simulink model "SUB_IoControl"  (R2018b)
settings: Solver=VariableStepDiscrete  StartTime=0.0  StopTime=10  RelTol=1e-3
PreLoadFcn:
  | if(exist('MBDS_ModelCallback', 'file'))
  |    MBDS_ModelCallback('PreLoad');
  | end
PostLoadFcn:
  | if(exist('MBDS_ModelCallback', 'file'))
  |    MBDS_ModelCallback('PostLoad');
  | end
InitFcn:
  | if(exist('MBDS_ModelCallback', 'file'))
  |    MBDS_ModelCallback('Init');
  | end
StartFcn:
  | if(exist('MBDS_ModelCallback', 'file'))
  |    MBDS_ModelCallback('Start');
  | end
StopFcn:
  | if(exist('MBDS_ModelCallback', 'file'))
  |    MBDS_ModelCallback('Stop');
  | end
undefined symbols (not defined in the file): sigbuilder_block
libraries: KIBES_Signal x742, MBDS_Modules x38, simulink x1
(part 7 of 8)

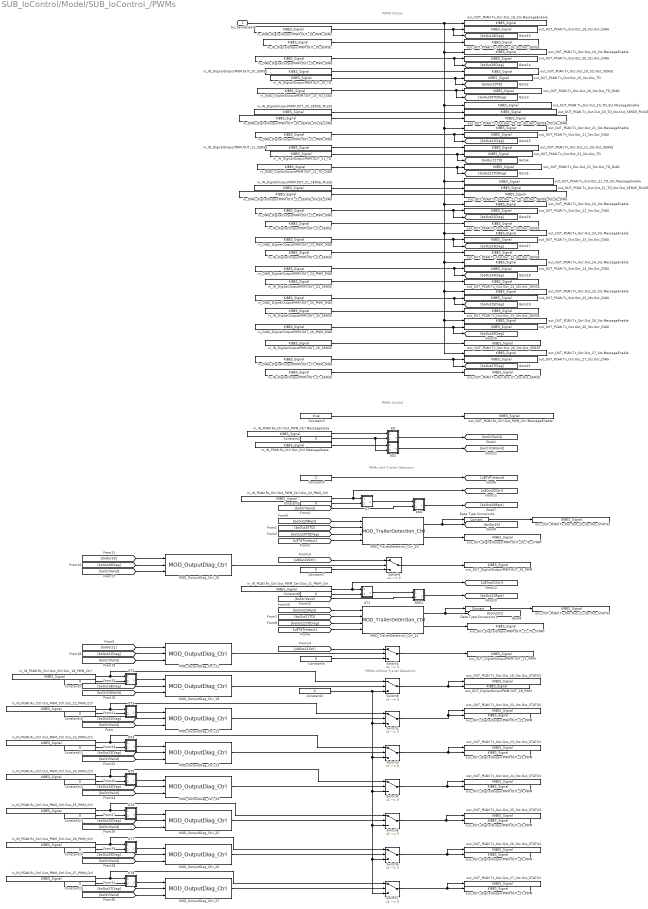
== system SUB_IoControl/Model/SUB_IoControl_/PWMs ==
  note: PWMs Control
  note: PWMs Status
  note: PWMs with Trailer Detection
  note: PWMs without Trailer Detection
  bo_SendEnable : Inport
  AND : Subsystem  InitFcn=|  mask(AND){MBDS_LibraryBlock=on, BitwiseMode=off, Inputs=2, UseBitMask=off, BitMask='A7', OutDataTypeStr=Inherit: Inherit via back propagation, MBDS_BlockVersion=08.20.02}
      | if(exist('MBDS_BlockCallback', 'file'))
      |    MBDS_BlockCallback('Update', gcb);
      | end
      mask prompts: MBDS_LibraryBlock "MBDS library block"; BitwiseMode "Use 'bitwise' mode"; Inputs "Number of input ports:"; UseBitMask "Use bit mask"; BitMask "Bit mask:"; OutDataTypeStr "Output data type:"; MBDS_BlockVersion "Version:"
      mask help: Logical or bitwise AND operator. For multiple inputs, operators are applied across the inputs. For a single input, operators are applied across the input vector. In bitwise mode a bit mask can be applied onto single input signals.
      mask init: same as SUB_IoControl/Outputs/AnalyseOutputs/And
      mask Help: eval(['open([workdir(''library_dir:''),''\Blockset\help\'',get_param(gcb,''MaskType''),''.html''])'])
      mask Callback BitwiseMode:
      | if(exist('MBDS_BlockCallback', 'file'))
      |    MBDS_BlockCallback('BitwiseMode', gcb);
      | end
      mask Callback Inputs:
      | if(exist('MBDS_BlockCallback', 'file'))
      |    MBDS_BlockCallback('Inputs', gcb);
      | end
      mask Callback UseBitMask:
      | if(exist('MBDS_BlockCallback', 'file'))
      |    MBDS_BlockCallback('UseBitMask', gcb);
      | end
      mask Callback BitMask:
      | if(exist('MBDS_BlockCallback', 'file'))
      |    MBDS_BlockCallback('BitMask', gcb);
      | end
      mask TypeOptions OutDataTypeStr: Inherit: Inherit via back propagation | int8 | uint8 | int16 | uint16 | int32 | uint32 | boolean
      mask Callback OutDataTypeStr:
      | % Adopt Value
      | if(exist('MBDS_BlockCallback', 'file'))
      |    MBDS_BlockCallback('OutDataTypeStr', gcb);
      | end
      mask DialogControl ParameterTabVar0 Prompt: Main
      mask DialogControl ParameterTabVar01 Prompt: Signal Attributes
      mask DialogControl ParameterTabVar012 Prompt: Version
      mask Display:
      | % Show icon or block text
      | if(UseBitMask)
      |    if(isnumeric(BitMask))
      |       BitMaskString = ['0x',dec2hex(floor(BitMask))];
      |    elseif(ischar(BitMask))
      |       BitMaskString = ['0x',upper(BitMask)];
      |    else
      |       BitMaskString = '???';
      |    end
      |    disp(sprintf(['AND\n', BitMaskString]))
      | else
      |    disp('AND')
      | end
  AND1 : Subsystem  InitFcn=|  mask(AND){MBDS_LibraryBlock=on, BitwiseMode=off, Inputs=2, UseBitMask=off, BitMask='A7', OutDataTypeStr=Inherit: Inherit via back propagation, MBDS_BlockVersion=08.20.02}
      | if(exist('MBDS_BlockCallback', 'file'))
      |    MBDS_BlockCallback('Update', gcb);
      | end
      mask prompts: MBDS_LibraryBlock "MBDS library block"; BitwiseMode "Use 'bitwise' mode"; Inputs "Number of input ports:"; UseBitMask "Use bit mask"; BitMask "Bit mask:"; OutDataTypeStr "Output data type:"; MBDS_BlockVersion "Version:"
      mask help: Logical or bitwise AND operator. For multiple inputs, operators are applied across the inputs. For a single input, operators are applied across the input vector. In bitwise mode a bit mask can be applied onto single input signals.
      mask init: same as SUB_IoControl/Outputs/AnalyseOutputs/And
      mask Help: eval(['open([workdir(''library_dir:''),''\Blockset\help\'',get_param(gcb,''MaskType''),''.html''])'])
      mask Callback BitwiseMode:
      | if(exist('MBDS_BlockCallback', 'file'))
      |    MBDS_BlockCallback('BitwiseMode', gcb);
      | end
      mask Callback Inputs:
      | if(exist('MBDS_BlockCallback', 'file'))
      |    MBDS_BlockCallback('Inputs', gcb);
      | end
      mask Callback UseBitMask:
      | if(exist('MBDS_BlockCallback', 'file'))
      |    MBDS_BlockCallback('UseBitMask', gcb);
      | end
      mask Callback BitMask:
      | if(exist('MBDS_BlockCallback', 'file'))
      |    MBDS_BlockCallback('BitMask', gcb);
      | end
      mask TypeOptions OutDataTypeStr: Inherit: Inherit via back propagation | int8 | uint8 | int16 | uint16 | int32 | uint32 | boolean
      mask Callback OutDataTypeStr:
      | % Adopt Value
      | if(exist('MBDS_BlockCallback', 'file'))
      |    MBDS_BlockCallback('OutDataTypeStr', gcb);
      | end
      mask DialogControl ParameterTabVar0 Prompt: Main
      mask DialogControl ParameterTabVar01 Prompt: Signal Attributes
      mask DialogControl ParameterTabVar012 Prompt: Version
      mask Display:
      | % Show icon or block text
      | if(UseBitMask)
      |    if(isnumeric(BitMask))
      |       BitMaskString = ['0x',dec2hex(floor(BitMask))];
      |    elseif(ischar(BitMask))
      |       BitMaskString = ['0x',upper(BitMask)];
      |    else
      |       BitMaskString = '???';
      |    end
      |    disp(sprintf(['AND\n', BitMaskString]))
      | else
      |    disp('AND')
      | end
  Constant1 : Constant  InitFcn=|  Value=0  OutDataTypeStr=uint16
      | if(exist('MBDS_BlockCallback', 'file'))
      |    MBDS_BlockCallback('Update', gcb);  
      | end
  Constant10 : Constant  InitFcn=|  Value=0  OutDataTypeStr=uint8
      | if(exist('MBDS_BlockCallback', 'file'))
      |    MBDS_BlockCallback('Update', gcb);  
      | end
  Constant11 : Constant  InitFcn=|  Value=0  OutDataTypeStr=uint8
      | if(exist('MBDS_BlockCallback', 'file'))
      |    MBDS_BlockCallback('Update', gcb);  
      | end
  Constant12 : Constant  InitFcn=|  Value=0  OutDataTypeStr=uint8
      | if(exist('MBDS_BlockCallback', 'file'))
      |    MBDS_BlockCallback('Update', gcb);  
      | end
  Constant13 : Constant  InitFcn=|  Value=0  OutDataTypeStr=uint8
      | if(exist('MBDS_BlockCallback', 'file'))
      |    MBDS_BlockCallback('Update', gcb);  
      | end
  Constant14 : Constant  InitFcn=|  Value=0  OutDataTypeStr=uint8
      | if(exist('MBDS_BlockCallback', 'file'))
      |    MBDS_BlockCallback('Update', gcb);  
      | end
  Constant15 : Constant  InitFcn=|  Value=0  OutDataTypeStr=uint8
      | if(exist('MBDS_BlockCallback', 'file'))
      |    MBDS_BlockCallback('Update', gcb);  
      | end
  Constant2 : Constant  InitFcn=|  Value=0  OutDataTypeStr=uint16
      | if(exist('MBDS_BlockCallback', 'file'))
      |    MBDS_BlockCallback('Update', gcb);  
      | end
  Constant3 : Constant  InitFcn=|  Value=true  OutDataTypeStr=boolean
      | if(exist('MBDS_BlockCallback', 'file'))
      |    MBDS_BlockCallback('Update', gcb);  
      | end
  Constant4 : Constant  InitFcn=|  Value=2  OutDataTypeStr=uint8
      | if(exist('MBDS_BlockCallback', 'file'))
      |    MBDS_BlockCallback('Update', gcb);  
      | end
  Constant5 : Constant  InitFcn=|  Value=0  OutDataTypeStr=uint8
      | if(exist('MBDS_BlockCallback', 'file'))
      |    MBDS_BlockCallback('Update', gcb);  
      | end
  Constant6 : Constant  InitFcn=|  Value=0  OutDataTypeStr=uint16
      | if(exist('MBDS_BlockCallback', 'file'))
      |    MBDS_BlockCallback('Update', gcb);  
      | end
  Constant7 : Constant  InitFcn=|  Value=0  OutDataTypeStr=uint8
      | if(exist('MBDS_BlockCallback', 'file'))
      |    MBDS_BlockCallback('Update', gcb);  
      | end
  Constant8 : Constant  InitFcn=|  Value=0  OutDataTypeStr=uint8
      | if(exist('MBDS_BlockCallback', 'file'))
      |    MBDS_BlockCallback('Update', gcb);  
      | end
  Constant9 : Constant  InitFcn=|  Value=0  OutDataTypeStr=uint8
      | if(exist('MBDS_BlockCallback', 'file'))
      |    MBDS_BlockCallback('Update', gcb);  
      | end
  Data Type Conversion : DataTypeConversion  InitFcn=|  SaturateOnIntegerOverflow=on
      | try
      |    MBDS_BlockCallback('Update', gcb);
      | end
      settings: AttributesFormatString=Saturate: %<SaturateOnIntegerOverflow>
  Data Type Conversion1 : DataTypeConversion  InitFcn=|  SaturateOnIntegerOverflow=on
      | try
      |    MBDS_BlockCallback('Update', gcb);
      | end
      settings: AttributesFormatString=Saturate: %<SaturateOnIntegerOverflow>
  EQ : Subsystem  InitFcn=|  mask(EQ){MBDS_LibraryBlock=on, InputSameDT=on, MBDS_BlockVersion=08.20.02}
      | if(exist('MBDS_BlockCallback', 'file'))
      |    MBDS_BlockCallback('Update', gcb);
      | end
      mask prompts: MBDS_LibraryBlock "MBDS library block"; InputSameDT "Require all inputs to have the same data type"; MBDS_BlockVersion "Block version:"
      mask help: The block compares if both input signals are equal.
      mask init: same as SUB_IoControl/Outputs/AnalyseOutputs/And
      mask Help: eval(['open([workdir(''library_dir:''),''\Blockset\help\'',get_param(gcb,''MaskType''),''.html''])'])
      mask Callback InputSameDT:
      | % Adopt value
      | if(exist('MBDS_BlockCallback', 'file'))
      |    MBDS_BlockCallback('InputSameDT', gcb);
      | end
      mask DialogControl ParameterTabVar0 Prompt: Signal Attributes
      mask DialogControl ParameterTabVar01 Prompt: Version
      mask Display:
      | % Show icon or block text
      | if(exist('MBDS_BlockCallback', 'file'))
      |    image(imread('EQ.tif','tif'),[0.35,0.35,0.355,0.25])
      |    disp('')
      | else
      |    disp(sprintf('=='));
      | end
  EQ1 : Subsystem  InitFcn=|  mask(EQ){MBDS_LibraryBlock=on, InputSameDT=on, MBDS_BlockVersion=08.20.02}
      | if(exist('MBDS_BlockCallback', 'file'))
      |    MBDS_BlockCallback('Update', gcb);
      | end
      mask prompts: MBDS_LibraryBlock "MBDS library block"; InputSameDT "Require all inputs to have the same data type"; MBDS_BlockVersion "Block version:"
      mask help: The block compares if both input signals are equal.
      mask init: same as SUB_IoControl/Outputs/AnalyseOutputs/And
      mask Help: eval(['open([workdir(''library_dir:''),''\Blockset\help\'',get_param(gcb,''MaskType''),''.html''])'])
      mask Callback InputSameDT:
      | % Adopt value
      | if(exist('MBDS_BlockCallback', 'file'))
      |    MBDS_BlockCallback('InputSameDT', gcb);
      | end
      mask DialogControl ParameterTabVar0 Prompt: Signal Attributes
      mask DialogControl ParameterTabVar01 Prompt: Version
      mask Display:
      | % Show icon or block text
      | if(exist('MBDS_BlockCallback', 'file'))
      |    image(imread('EQ.tif','tif'),[0.35,0.35,0.355,0.25])
      |    disp('')
      | else
      |    disp(sprintf('=='));
      | end
  GT : Subsystem  InitFcn=|  mask(GT){MBDS_LibraryBlock=on, InputSameDT=on, MBDS_BlockVersion=08.20.02}
      | if(exist('MBDS_BlockCallback', 'file'))
      |    MBDS_BlockCallback('Update', gcb);
      | end
      mask prompts: MBDS_LibraryBlock "MBDS library block"; InputSameDT "Require all inputs to have the same data type"; MBDS_BlockVersion "Block version:"
      mask help: The block compares if the first input signal is greater than the second input signal.
      mask init: same as SUB_IoControl/Outputs/AnalyseOutputs/And
      mask Help: eval(['open([workdir(''library_dir:''),''\Blockset\help\'',get_param(gcb,''MaskType''),''.html''])'])
      mask Callback InputSameDT:
      | % Adopt value
      | if(exist('MBDS_BlockCallback', 'file'))
      |    MBDS_BlockCallback('InputSameDT', gcb);
      | end
      mask DialogControl ParameterTabVar0 Prompt: Signal Attributes
      mask DialogControl ParameterTabVar01 Prompt: Version
      mask Display:
      | % Show icon or block text
      | if(exist('MBDS_BlockCallback', 'file'))
      |    image(imread('GT.tif','tif'),[0.33,0.33,0.37,0.37])
      |    disp('')
      | else
      |    disp(sprintf('>'));
      | end
  GT1 : Subsystem  InitFcn=|  mask(GT){MBDS_LibraryBlock=on, InputSameDT=on, MBDS_BlockVersion=08.20.02}
      | if(exist('MBDS_BlockCallback', 'file'))
      |    MBDS_BlockCallback('Update', gcb);
      | end
      mask prompts: MBDS_LibraryBlock "MBDS library block"; InputSameDT "Require all inputs to have the same data type"; MBDS_BlockVersion "Block version:"
      mask help: The block compares if the first input signal is greater than the second input signal.
      mask init: same as SUB_IoControl/Outputs/AnalyseOutputs/And
      mask Help: eval(['open([workdir(''library_dir:''),''\Blockset\help\'',get_param(gcb,''MaskType''),''.html''])'])
      mask Callback InputSameDT:
      | % Adopt value
      | if(exist('MBDS_BlockCallback', 'file'))
      |    MBDS_BlockCallback('InputSameDT', gcb);
      | end
      mask DialogControl ParameterTabVar0 Prompt: Signal Attributes
      mask DialogControl ParameterTabVar01 Prompt: Version
      mask Display:
      | % Show icon or block text
      | if(exist('MBDS_BlockCallback', 'file'))
      |    image(imread('GT.tif','tif'),[0.33,0.33,0.37,0.37])
      |    disp('')
      | else
      |    disp(sprintf('>'));
      | end
  GT2 : Subsystem  InitFcn=|  mask(GT){MBDS_LibraryBlock=on, InputSameDT=on, MBDS_BlockVersion=08.20.02}
      | if(exist('MBDS_BlockCallback', 'file'))
      |    MBDS_BlockCallback('Update', gcb);
      | end
      mask prompts: MBDS_LibraryBlock "MBDS library block"; InputSameDT "Require all inputs to have the same data type"; MBDS_BlockVersion "Block version:"
      mask help: The block compares if the first input signal is greater than the second input signal.
      mask init: same as SUB_IoControl/Outputs/AnalyseOutputs/And
      mask Help: eval(['open([workdir(''library_dir:''),''\Blockset\help\'',get_param(gcb,''MaskType''),''.html''])'])
      mask Callback InputSameDT:
      | % Adopt value
      | if(exist('MBDS_BlockCallback', 'file'))
      |    MBDS_BlockCallback('InputSameDT', gcb);
      | end
      mask DialogControl ParameterTabVar0 Prompt: Signal Attributes
      mask DialogControl ParameterTabVar01 Prompt: Version
      mask Display:
      | % Show icon or block text
      | if(exist('MBDS_BlockCallback', 'file'))
      |    image(imread('GT.tif','tif'),[0.33,0.33,0.37,0.37])
      |    disp('')
      | else
      |    disp(sprintf('>'));
      | end
  GT3 : Subsystem  InitFcn=|  mask(GT){MBDS_LibraryBlock=on, InputSameDT=on, MBDS_BlockVersion=08.20.02}
      | if(exist('MBDS_BlockCallback', 'file'))
      |    MBDS_BlockCallback('Update', gcb);
      | end
      mask prompts: MBDS_LibraryBlock "MBDS library block"; InputSameDT "Require all inputs to have the same data type"; MBDS_BlockVersion "Block version:"
      mask help: The block compares if the first input signal is greater than the second input signal.
      mask init: same as SUB_IoControl/Outputs/AnalyseOutputs/And
      mask Help: eval(['open([workdir(''library_dir:''),''\Blockset\help\'',get_param(gcb,''MaskType''),''.html''])'])
      mask Callback InputSameDT:
      | % Adopt value
      | if(exist('MBDS_BlockCallback', 'file'))
      |    MBDS_BlockCallback('InputSameDT', gcb);
      | end
      mask DialogControl ParameterTabVar0 Prompt: Signal Attributes
      mask DialogControl ParameterTabVar01 Prompt: Version
      mask Display:
      | % Show icon or block text
      | if(exist('MBDS_BlockCallback', 'file'))
      |    image(imread('GT.tif','tif'),[0.33,0.33,0.37,0.37])
      |    disp('')
      | else
      |    disp(sprintf('>'));
      | end
  GT4 : Subsystem  InitFcn=|  mask(GT){MBDS_LibraryBlock=on, InputSameDT=on, MBDS_BlockVersion=08.20.02}
      | if(exist('MBDS_BlockCallback', 'file'))
      |    MBDS_BlockCallback('Update', gcb);
      | end
      mask prompts: MBDS_LibraryBlock "MBDS library block"; InputSameDT "Require all inputs to have the same data type"; MBDS_BlockVersion "Block version:"
      mask help: The block compares if the first input signal is greater than the second input signal.
      mask init: same as SUB_IoControl/Outputs/AnalyseOutputs/And
      mask Help: eval(['open([workdir(''library_dir:''),''\Blockset\help\'',get_param(gcb,''MaskType''),''.html''])'])
      mask Callback InputSameDT:
      | % Adopt value
      | if(exist('MBDS_BlockCallback', 'file'))
      |    MBDS_BlockCallback('InputSameDT', gcb);
      | end
      mask DialogControl ParameterTabVar0 Prompt: Signal Attributes
      mask DialogControl ParameterTabVar01 Prompt: Version
      mask Display:
      | % Show icon or block text
      | if(exist('MBDS_BlockCallback', 'file'))
      |    image(imread('GT.tif','tif'),[0.33,0.33,0.37,0.37])
      |    disp('')
      | else
      |    disp(sprintf('>'));
      | end
  GT5 : Subsystem  InitFcn=|  mask(GT){MBDS_LibraryBlock=on, InputSameDT=on, MBDS_BlockVersion=08.20.02}
      | if(exist('MBDS_BlockCallback', 'file'))
      |    MBDS_BlockCallback('Update', gcb);
      | end
      mask prompts: MBDS_LibraryBlock "MBDS library block"; InputSameDT "Require all inputs to have the same data type"; MBDS_BlockVersion "Block version:"
      mask help: The block compares if the first input signal is greater than the second input signal.
      mask init: same as SUB_IoControl/Outputs/AnalyseOutputs/And
      mask Help: eval(['open([workdir(''library_dir:''),''\Blockset\help\'',get_param(gcb,''MaskType''),''.html''])'])
      mask Callback InputSameDT:
      | % Adopt value
      | if(exist('MBDS_BlockCallback', 'file'))
      |    MBDS_BlockCallback('InputSameDT', gcb);
      | end
      mask DialogControl ParameterTabVar0 Prompt: Signal Attributes
      mask DialogControl ParameterTabVar01 Prompt: Version
      mask Display:
      | % Show icon or block text
      | if(exist('MBDS_BlockCallback', 'file'))
      |    image(imread('GT.tif','tif'),[0.33,0.33,0.37,0.37])
      |    disp('')
      | else
      |    disp(sprintf('>'));
      | end
  GT6 : Subsystem  InitFcn=|  mask(GT){MBDS_LibraryBlock=on, InputSameDT=on, MBDS_BlockVersion=08.20.02}
      | if(exist('MBDS_BlockCallback', 'file'))
      |    MBDS_BlockCallback('Update', gcb);
      | end
      mask prompts: MBDS_LibraryBlock "MBDS library block"; InputSameDT "Require all inputs to have the same data type"; MBDS_BlockVersion "Block version:"
      mask help: The block compares if the first input signal is greater than the second input signal.
      mask init: same as SUB_IoControl/Outputs/AnalyseOutputs/And
      mask Help: eval(['open([workdir(''library_dir:''),''\Blockset\help\'',get_param(gcb,''MaskType''),''.html''])'])
      mask Callback InputSameDT:
      | % Adopt value
      | if(exist('MBDS_BlockCallback', 'file'))
      |    MBDS_BlockCallback('InputSameDT', gcb);
      | end
      mask DialogControl ParameterTabVar0 Prompt: Signal Attributes
      mask DialogControl ParameterTabVar01 Prompt: Version
      mask Display:
      | % Show icon or block text
      | if(exist('MBDS_BlockCallback', 'file'))
      |    image(imread('GT.tif','tif'),[0.33,0.33,0.37,0.37])
      |    disp('')
      | else
      |    disp(sprintf('>'));
      | end
  GT7 : Subsystem  InitFcn=|  mask(GT){MBDS_LibraryBlock=on, InputSameDT=on, MBDS_BlockVersion=08.20.02}
      | if(exist('MBDS_BlockCallback', 'file'))
      |    MBDS_BlockCallback('Update', gcb);
      | end
      mask prompts: MBDS_LibraryBlock "MBDS library block"; InputSameDT "Require all inputs to have the same data type"; MBDS_BlockVersion "Block version:"
      mask help: The block compares if the first input signal is greater than the second input signal.
      mask init: same as SUB_IoControl/Outputs/AnalyseOutputs/And
      mask Help: eval(['open([workdir(''library_dir:''),''\Blockset\help\'',get_param(gcb,''MaskType''),''.html''])'])
      mask Callback InputSameDT:
      | % Adopt value
      | if(exist('MBDS_BlockCallback', 'file'))
      |    MBDS_BlockCallback('InputSameDT', gcb);
      | end
      mask DialogControl ParameterTabVar0 Prompt: Signal Attributes
      mask DialogControl ParameterTabVar01 Prompt: Version
      mask Display:
      | % Show icon or block text
      | if(exist('MBDS_BlockCallback', 'file'))
      |    image(imread('GT.tif','tif'),[0.33,0.33,0.37,0.37])
      |    disp('')
      | else
      |    disp(sprintf('>'));
      | end
  GT8 : Subsystem  InitFcn=|  mask(GT){MBDS_LibraryBlock=on, InputSameDT=on, MBDS_BlockVersion=08.20.02}
      | if(exist('MBDS_BlockCallback', 'file'))
      |    MBDS_BlockCallback('Update', gcb);
      | end
      mask prompts: MBDS_LibraryBlock "MBDS library block"; InputSameDT "Require all inputs to have the same data type"; MBDS_BlockVersion "Block version:"
      mask help: The block compares if the first input signal is greater than the second input signal.
      mask init: same as SUB_IoControl/Outputs/AnalyseOutputs/And
      mask Help: eval(['open([workdir(''library_dir:''),''\Blockset\help\'',get_param(gcb,''MaskType''),''.html''])'])
      mask Callback InputSameDT:
      | % Adopt value
      | if(exist('MBDS_BlockCallback', 'file'))
      |    MBDS_BlockCallback('InputSameDT', gcb);
      | end
      mask DialogControl ParameterTabVar0 Prompt: Signal Attributes
      mask DialogControl ParameterTabVar01 Prompt: Version
      mask Display:
      | % Show icon or block text
      | if(exist('MBDS_BlockCallback', 'file'))
      |    image(imread('GT.tif','tif'),[0.33,0.33,0.37,0.37])
      |    disp('')
      | else
      |    disp(sprintf('>'));
      | end
  MOD_OutputDiag_Ctrl_{18,20..27} (9 alike) : MBDS_Modules/MOD_OutputDiag_Ctrl  Description=Controls output based on diagnostic signal  MBDS_ElementType=Module  MBDS_WorkStatus=In Work  MBDS_LastModified=2021-03-24-14:11:54
      settings: SourceProductName=MBDS Project Library
  MOD_TrailerDetection_Ctrl_20 : MBDS_Modules/MOD_TrailerDetection_Ctrl  Description=Control outputs with Trailer detection hardware.  MBDS_ElementType=Module  MBDS_WorkStatus=In Work  MBDS_LastModified=2020-12-28-09:09:43
      settings: SourceProductName=MBDS Project Library
  MOD_TrailerDetection_Ctrl_21 : MBDS_Modules/MOD_TrailerDetection_Ctrl  Description=Control outputs with Trailer detection hardware.  MBDS_ElementType=Module  MBDS_WorkStatus=In Work  MBDS_LastModified=2020-12-28-09:09:43
      settings: SourceProductName=MBDS Project Library
  Switch1 : Switch  InitFcn=|  Criteria=u2 ~= 0  OutDataTypeStr=Inherit: Inherit via back propagation  mask(Switch){MBDS_LibraryBlock=on, OutDataTypeStr_=Inherit: Inherit via back propagation, SaturateOnIntegerOverflow_=off, InputSameDT_=off, MBDS_BlockVersion=08.20.02}
      | if(exist('MBDS_BlockCallback', 'file'))
      |    MBDS_BlockCallback('Update', gcb);  
      | end
      mask prompts: MBDS_LibraryBlock "MBDS library block"; OutDataTypeStr_ "Output data type:"; SaturateOnIntegerOverflow_ "Saturate on integer overflow"; InputSameDT_ "Require all inputs to have the same data type"; MBDS_BlockVersion "Block version:"
      mask help: Pass through input 1 when input 2 is not equal to zero; otherwise pass through input 3. The inputs are numbered top to bottom (or left to right). The first and third input ports are data ports, and the second input port is the control port.
      mask init: same as SUB_IoControl/Outputs/AnalyseOutputs/And
      mask Help: eval(['open([workdir(''library_dir:''),''\Blockset\help\'',get_param(gcb,''MaskType''),''.html''])'])
      mask TypeOptions OutDataTypeStr_: Inherit: Inherit via back propagation | single | int8 | uint8 | int16 | uint16 | int32 | uint32
      mask DialogControl ParameterTabVar0 Prompt: Signal Attributes
      mask DialogControl ParameterTabVar01 Prompt: Version
  Switch2 : Switch  InitFcn=|  Criteria=u2 ~= 0  OutDataTypeStr=Inherit: Inherit via back propagation  mask(Switch){MBDS_LibraryBlock=on, OutDataTypeStr_=Inherit: Inherit via back propagation, SaturateOnIntegerOverflow_=off, InputSameDT_=off, MBDS_BlockVersion=08.20.02}
      | if(exist('MBDS_BlockCallback', 'file'))
      |    MBDS_BlockCallback('Update', gcb);  
      | end
      mask prompts: MBDS_LibraryBlock "MBDS library block"; OutDataTypeStr_ "Output data type:"; SaturateOnIntegerOverflow_ "Saturate on integer overflow"; InputSameDT_ "Require all inputs to have the same data type"; MBDS_BlockVersion "Block version:"
      mask help: Pass through input 1 when input 2 is not equal to zero; otherwise pass through input 3. The inputs are numbered top to bottom (or left to right). The first and third input ports are data ports, and the second input port is the control port.
      mask init: same as SUB_IoControl/Outputs/AnalyseOutputs/And
      mask Help: eval(['open([workdir(''library_dir:''),''\Blockset\help\'',get_param(gcb,''MaskType''),''.html''])'])
      mask TypeOptions OutDataTypeStr_: Inherit: Inherit via back propagation | single | int8 | uint8 | int16 | uint16 | int32 | uint32
      mask DialogControl ParameterTabVar0 Prompt: Signal Attributes
      mask DialogControl ParameterTabVar01 Prompt: Version
  Switch3 : Switch  InitFcn=|  Criteria=u2 ~= 0  OutDataTypeStr=Inherit: Inherit via back propagation  mask(Switch){MBDS_LibraryBlock=on, OutDataTypeStr_=Inherit: Inherit via back propagation, SaturateOnIntegerOverflow_=off, InputSameDT_=off, MBDS_BlockVersion=08.20.02}
      | if(exist('MBDS_BlockCallback', 'file'))
      |    MBDS_BlockCallback('Update', gcb);  
      | end
      mask prompts: MBDS_LibraryBlock "MBDS library block"; OutDataTypeStr_ "Output data type:"; SaturateOnIntegerOverflow_ "Saturate on integer overflow"; InputSameDT_ "Require all inputs to have the same data type"; MBDS_BlockVersion "Block version:"
      mask help: Pass through input 1 when input 2 is not equal to zero; otherwise pass through input 3. The inputs are numbered top to bottom (or left to right). The first and third input ports are data ports, and the second input port is the control port.
      mask init: same as SUB_IoControl/Outputs/AnalyseOutputs/And
      mask Help: eval(['open([workdir(''library_dir:''),''\Blockset\help\'',get_param(gcb,''MaskType''),''.html''])'])
      mask TypeOptions OutDataTypeStr_: Inherit: Inherit via back propagation | single | int8 | uint8 | int16 | uint16 | int32 | uint32
      mask DialogControl ParameterTabVar0 Prompt: Signal Attributes
      mask DialogControl ParameterTabVar01 Prompt: Version
  Switch4 : Switch  InitFcn=|  Criteria=u2 ~= 0  OutDataTypeStr=Inherit: Inherit via back propagation  mask(Switch){MBDS_LibraryBlock=on, OutDataTypeStr_=Inherit: Inherit via back propagation, SaturateOnIntegerOverflow_=off, InputSameDT_=off, MBDS_BlockVersion=08.20.02}
      | if(exist('MBDS_BlockCallback', 'file'))
      |    MBDS_BlockCallback('Update', gcb);  
      | end
      mask prompts: MBDS_LibraryBlock "MBDS library block"; OutDataTypeStr_ "Output data type:"; SaturateOnIntegerOverflow_ "Saturate on integer overflow"; InputSameDT_ "Require all inputs to have the same data type"; MBDS_BlockVersion "Block version:"
      mask help: Pass through input 1 when input 2 is not equal to zero; otherwise pass through input 3. The inputs are numbered top to bottom (or left to right). The first and third input ports are data ports, and the second input port is the control port.
      mask init: same as SUB_IoControl/Outputs/AnalyseOutputs/And
      mask Help: eval(['open([workdir(''library_dir:''),''\Blockset\help\'',get_param(gcb,''MaskType''),''.html''])'])
      mask TypeOptions OutDataTypeStr_: Inherit: Inherit via back propagation | single | int8 | uint8 | int16 | uint16 | int32 | uint32
      mask DialogControl ParameterTabVar0 Prompt: Signal Attributes
      mask DialogControl ParameterTabVar01 Prompt: Version
  Switch5 : Switch  InitFcn=|  Criteria=u2 ~= 0  OutDataTypeStr=Inherit: Inherit via back propagation  mask(Switch){MBDS_LibraryBlock=on, OutDataTypeStr_=Inherit: Inherit via back propagation, SaturateOnIntegerOverflow_=off, InputSameDT_=off, MBDS_BlockVersion=08.20.02}
      | if(exist('MBDS_BlockCallback', 'file'))
      |    MBDS_BlockCallback('Update', gcb);  
      | end
      mask prompts: MBDS_LibraryBlock "MBDS library block"; OutDataTypeStr_ "Output data type:"; SaturateOnIntegerOverflow_ "Saturate on integer overflow"; InputSameDT_ "Require all inputs to have the same data type"; MBDS_BlockVersion "Block version:"
      mask help: Pass through input 1 when input 2 is not equal to zero; otherwise pass through input 3. The inputs are numbered top to bottom (or left to right). The first and third input ports are data ports, and the second input port is the control port.
      mask init: same as SUB_IoControl/Outputs/AnalyseOutputs/And
      mask Help: eval(['open([workdir(''library_dir:''),''\Blockset\help\'',get_param(gcb,''MaskType''),''.html''])'])
      mask TypeOptions OutDataTypeStr_: Inherit: Inherit via back propagation | single | int8 | uint8 | int16 | uint16 | int32 | uint32
      mask DialogControl ParameterTabVar0 Prompt: Signal Attributes
      mask DialogControl ParameterTabVar01 Prompt: Version
  Switch6 : Switch  InitFcn=|  Criteria=u2 ~= 0  OutDataTypeStr=Inherit: Inherit via back propagation  mask(Switch){MBDS_LibraryBlock=on, OutDataTypeStr_=Inherit: Inherit via back propagation, SaturateOnIntegerOverflow_=off, InputSameDT_=off, MBDS_BlockVersion=08.20.02}
      | if(exist('MBDS_BlockCallback', 'file'))
      |    MBDS_BlockCallback('Update', gcb);  
      | end
      mask prompts: MBDS_LibraryBlock "MBDS library block"; OutDataTypeStr_ "Output data type:"; SaturateOnIntegerOverflow_ "Saturate on integer overflow"; InputSameDT_ "Require all inputs to have the same data type"; MBDS_BlockVersion "Block version:"
      mask help: Pass through input 1 when input 2 is not equal to zero; otherwise pass through input 3. The inputs are numbered top to bottom (or left to right). The first and third input ports are data ports, and the second input port is the control port.
      mask init: same as SUB_IoControl/Outputs/AnalyseOutputs/And
      mask Help: eval(['open([workdir(''library_dir:''),''\Blockset\help\'',get_param(gcb,''MaskType''),''.html''])'])
      mask TypeOptions OutDataTypeStr_: Inherit: Inherit via back propagation | single | int8 | uint8 | int16 | uint16 | int32 | uint32
      mask DialogControl ParameterTabVar0 Prompt: Signal Attributes
      mask DialogControl ParameterTabVar01 Prompt: Version
  Switch7 : Switch  InitFcn=|  Criteria=u2 ~= 0  OutDataTypeStr=Inherit: Inherit via back propagation  mask(Switch){MBDS_LibraryBlock=on, OutDataTypeStr_=Inherit: Inherit via back propagation, SaturateOnIntegerOverflow_=off, InputSameDT_=off, MBDS_BlockVersion=08.20.02}
      | if(exist('MBDS_BlockCallback', 'file'))
      |    MBDS_BlockCallback('Update', gcb);  
      | end
      mask prompts: MBDS_LibraryBlock "MBDS library block"; OutDataTypeStr_ "Output data type:"; SaturateOnIntegerOverflow_ "Saturate on integer overflow"; InputSameDT_ "Require all inputs to have the same data type"; MBDS_BlockVersion "Block version:"
      mask help: Pass through input 1 when input 2 is not equal to zero; otherwise pass through input 3. The inputs are numbered top to bottom (or left to right). The first and third input ports are data ports, and the second input port is the control port.
      mask init: same as SUB_IoControl/Outputs/AnalyseOutputs/And
      mask Help: eval(['open([workdir(''library_dir:''),''\Blockset\help\'',get_param(gcb,''MaskType''),''.html''])'])
      mask TypeOptions OutDataTypeStr_: Inherit: Inherit via back propagation | single | int8 | uint8 | int16 | uint16 | int32 | uint32
      mask DialogControl ParameterTabVar0 Prompt: Signal Attributes
      mask DialogControl ParameterTabVar01 Prompt: Version
  Switch8 : Switch  InitFcn=|  Criteria=u2 ~= 0  OutDataTypeStr=Inherit: Inherit via back propagation  mask(Switch){MBDS_LibraryBlock=on, OutDataTypeStr_=Inherit: Inherit via back propagation, SaturateOnIntegerOverflow_=off, InputSameDT_=off, MBDS_BlockVersion=08.20.02}
      | if(exist('MBDS_BlockCallback', 'file'))
      |    MBDS_BlockCallback('Update', gcb);  
      | end
      mask prompts: MBDS_LibraryBlock "MBDS library block"; OutDataTypeStr_ "Output data type:"; SaturateOnIntegerOverflow_ "Saturate on integer overflow"; InputSameDT_ "Require all inputs to have the same data type"; MBDS_BlockVersion "Block version:"
      mask help: Pass through input 1 when input 2 is not equal to zero; otherwise pass through input 3. The inputs are numbered top to bottom (or left to right). The first and third input ports are data ports, and the second input port is the control port.
      mask init: same as SUB_IoControl/Outputs/AnalyseOutputs/And
      mask Help: eval(['open([workdir(''library_dir:''),''\Blockset\help\'',get_param(gcb,''MaskType''),''.html''])'])
      mask TypeOptions OutDataTypeStr_: Inherit: Inherit via back propagation | single | int8 | uint8 | int16 | uint16 | int32 | uint32
      mask DialogControl ParameterTabVar0 Prompt: Signal Attributes
      mask DialogControl ParameterTabVar01 Prompt: Version
  Switch9 : Switch  InitFcn=|  Criteria=u2 ~= 0  OutDataTypeStr=Inherit: Inherit via back propagation  mask(Switch){MBDS_LibraryBlock=on, OutDataTypeStr_=Inherit: Inherit via back propagation, SaturateOnIntegerOverflow_=off, InputSameDT_=off, MBDS_BlockVersion=08.20.02}
      | if(exist('MBDS_BlockCallback', 'file'))
      |    MBDS_BlockCallback('Update', gcb);  
      | end
      mask prompts: MBDS_LibraryBlock "MBDS library block"; OutDataTypeStr_ "Output data type:"; SaturateOnIntegerOverflow_ "Saturate on integer overflow"; InputSameDT_ "Require all inputs to have the same data type"; MBDS_BlockVersion "Block version:"
      mask help: Pass through input 1 when input 2 is not equal to zero; otherwise pass through input 3. The inputs are numbered top to bottom (or left to right). The first and third input ports are data ports, and the second input port is the control port.
      mask init: same as SUB_IoControl/Outputs/AnalyseOutputs/And
      mask Help: eval(['open([workdir(''library_dir:''),''\Blockset\help\'',get_param(gcb,''MaskType''),''.html''])'])
      mask TypeOptions OutDataTypeStr_: Inherit: Inherit via back propagation | single | int8 | uint8 | int16 | uint16 | int32 | uint32
      mask DialogControl ParameterTabVar0 Prompt: Signal Attributes
      mask DialogControl ParameterTabVar01 Prompt: Version
  in_DIAG_DigitalOutputPWM.OUT_18_PWM_DIAG : KIBES_Signal/KIBES_Signal  MBDS_LibraryBlock=on  DatabaseKey=2283  SignalName=DIAG_DigitalOutputPWM.OUT_18_PWM_DIAG  SymbolName=DIAG_DigitalOutputPWM_OUT_18_PWM_DIAG_002283  DataType=uint16  Init=1  Slope=1  Bias=0  DataSize=1  fpDataType=uint16  BlockIOType=Inport  DeviceType=0
  in_DIAG_DigitalOutputPWM.OUT_20_PWM_DIAG : KIBES_Signal/KIBES_Signal  MBDS_LibraryBlock=on  DatabaseKey=779  SignalName=DIAG_DigitalOutputPWM.OUT_20_PWM_DIAG  SymbolName=DIAG_DigitalOutputPWM_OUT_20_PWM_DIAG_000779  DataType=uint16  Init=1  Slope=1  Bias=0  DataSize=1  fpDataType=uint16  BlockIOType=Inport  DeviceType=0
  in_DIAG_DigitalOutputPWM.OUT_20_SENSE_PULSE_DIAG : KIBES_Signal/KIBES_Signal  MBDS_LibraryBlock=on  DatabaseKey=2221  SignalName=DIAG_DigitalOutputPWM.OUT_20_SENSE_PULSE_DIAG  SymbolName=DIAG_DigitalOutputPWM_OUT_20_SENSE_PULSE_DIAG_002221  DataType=uint16  Init=1  Slope=1  Bias=0  DataSize=1  fpDataType=uint16  BlockIOType=Inport  DeviceType=0
  in_DIAG_DigitalOutputPWM.OUT_20_TD_DIAG : KIBES_Signal/KIBES_Signal  MBDS_LibraryBlock=on  DatabaseKey=784  SignalName=DIAG_DigitalOutputPWM.OUT_20_TD_DIAG  SymbolName=DIAG_DigitalOutputPWM_OUT_20_TD_DIAG_000784  DataType=uint16  Init=1  Slope=1  Bias=0  DataSize=1  fpDataType=uint16  BlockIOType=Inport  DeviceType=0
  in_DIAG_DigitalOutputPWM.OUT_21_PWM_DIAG : KIBES_Signal/KIBES_Signal  MBDS_LibraryBlock=on  DatabaseKey=787  SignalName=DIAG_DigitalOutputPWM.OUT_21_PWM_DIAG  SymbolName=DIAG_DigitalOutputPWM_OUT_21_PWM_DIAG_000787  DataType=uint16  Init=1  Slope=1  Bias=0  DataSize=1  fpDataType=uint16  BlockIOType=Inport  DeviceType=0
  in_DIAG_DigitalOutputPWM.OUT_21_SENSE_PULSE_DIAG : KIBES_Signal/KIBES_Signal  MBDS_LibraryBlock=on  DatabaseKey=2223  SignalName=DIAG_DigitalOutputPWM.OUT_21_SENSE_PULSE_DIAG  SymbolName=DIAG_DigitalOutputPWM_OUT_21_SENSE_PULSE_DIAG_002223  DataType=uint16  Init=1  Slope=1  Bias=0  DataSize=1  fpDataType=uint16  BlockIOType=Inport  DeviceType=0
  in_DIAG_DigitalOutputPWM.OUT_21_TD_DIAG : KIBES_Signal/KIBES_Signal  MBDS_LibraryBlock=on  DatabaseKey=792  SignalName=DIAG_DigitalOutputPWM.OUT_21_TD_DIAG  SymbolName=DIAG_DigitalOutputPWM_OUT_21_TD_DIAG_000792  DataType=uint16  Init=1  Slope=1  Bias=0  DataSize=1  fpDataType=uint16  BlockIOType=Inport  DeviceType=0
  in_DIAG_DigitalOutputPWM.OUT_22_PWM_DIAG : KIBES_Signal/KIBES_Signal  MBDS_LibraryBlock=on  DatabaseKey=767  SignalName=DIAG_DigitalOutputPWM.OUT_22_PWM_DIAG  SymbolName=DIAG_DigitalOutputPWM_OUT_22_PWM_DIAG_000767  DataType=uint16  Init=1  Slope=1  Bias=0  DataSize=1  fpDataType=uint16  BlockIOType=Inport  DeviceType=0
  in_DIAG_DigitalOutputPWM.OUT_23_PWM_DIAG : KIBES_Signal/KIBES_Signal  MBDS_LibraryBlock=on  DatabaseKey=770  SignalName=DIAG_DigitalOutputPWM.OUT_23_PWM_DIAG  SymbolName=DIAG_DigitalOutputPWM_OUT_23_PWM_DIAG_000770  DataType=uint16  Init=1  Slope=1  Bias=0  DataSize=1  fpDataType=uint16  BlockIOType=Inport  DeviceType=0
  in_DIAG_DigitalOutputPWM.OUT_24_PWM_DIAG : KIBES_Signal/KIBES_Signal  MBDS_LibraryBlock=on  DatabaseKey=773  SignalName=DIAG_DigitalOutputPWM.OUT_24_PWM_DIAG  SymbolName=DIAG_DigitalOutputPWM_OUT_24_PWM_DIAG_000773  DataType=uint16  Init=1  Slope=1  Bias=0  DataSize=1  fpDataType=uint16  BlockIOType=Inport  DeviceType=0
  in_DIAG_DigitalOutputPWM.OUT_25_PWM_DIAG : KIBES_Signal/KIBES_Signal  MBDS_LibraryBlock=on  DatabaseKey=776  SignalName=DIAG_DigitalOutputPWM.OUT_25_PWM_DIAG  SymbolName=DIAG_DigitalOutputPWM_OUT_25_PWM_DIAG_000776  DataType=uint16  Init=1  Slope=1  Bias=0  DataSize=1  fpDataType=uint16  BlockIOType=Inport  DeviceType=0
  in_DIAG_DigitalOutputPWM.OUT_26_PWM_DIAG : KIBES_Signal/KIBES_Signal  MBDS_LibraryBlock=on  DatabaseKey=794  SignalName=DIAG_DigitalOutputPWM.OUT_26_PWM_DIAG  SymbolName=DIAG_DigitalOutputPWM_OUT_26_PWM_DIAG_000794  DataType=uint16  Init=1  Slope=1  Bias=0  DataSize=1  fpDataType=uint16  BlockIOType=Inport  DeviceType=0
  in_DIAG_DigitalOutputPWM.OUT_27_PWM_DIAG : KIBES_Signal/KIBES_Signal  MBDS_LibraryBlock=on  DatabaseKey=797  SignalName=DIAG_DigitalOutputPWM.OUT_27_PWM_DIAG  SymbolName=DIAG_DigitalOutputPWM_OUT_27_PWM_DIAG_000797  DataType=uint16  Init=1  Slope=1  Bias=0  DataSize=1  fpDataType=uint16  BlockIOType=Inport  DeviceType=0
  in_IN_DigitalOutputPWM.OUT_18_SENSE : KIBES_Signal/KIBES_Signal  MBDS_LibraryBlock=on  DatabaseKey=2284  SignalName=IN_DigitalOutputPWM.OUT_18_SENSE  SymbolName=IN_DigitalOutputPWM_OUT_18_SENSE_002284  DataType=uint16  Init=0  Slope=1  Bias=0  DataSize=1  fpDataType=uint16  BlockIOType=Inport  DeviceType=0
  in_IN_DigitalOutputPWM.OUT_20_SENSE : KIBES_Signal/KIBES_Signal  MBDS_LibraryBlock=on  DatabaseKey=780  SignalName=IN_DigitalOutputPWM.OUT_20_SENSE  SymbolName=IN_DigitalOutputPWM_OUT_20_SENSE_000780  DataType=uint16  Init=0  Slope=1  Bias=0  DataSize=1  fpDataType=uint16  BlockIOType=Inport  DeviceType=0
  in_IN_DigitalOutputPWM.OUT_20_SENSE_PULSE : KIBES_Signal/KIBES_Signal  MBDS_LibraryBlock=on  DatabaseKey=2220  SignalName=IN_DigitalOutputPWM.OUT_20_SENSE_PULSE  SymbolName=IN_DigitalOutputPWM_OUT_20_SENSE_PULSE_002220  DataType=uint16  Init=0  Slope=1  Bias=0  DataSize=1  fpDataType=uint16  BlockIOType=Inport  DeviceType=0
  in_IN_DigitalOutputPWM.OUT_20_TD : KIBES_Signal/KIBES_Signal  MBDS_LibraryBlock=on  DatabaseKey=783  SignalName=IN_DigitalOutputPWM.OUT_20_TD  SymbolName=IN_DigitalOutputPWM_OUT_20_TD_000783  DataType=boolean  Init=0  Slope=1  Bias=0  DataSize=1  fpDataType=boolean  BlockIOType=Inport  DeviceType=0
  in_IN_DigitalOutputPWM.OUT_21_SENSE : KIBES_Signal/KIBES_Signal  MBDS_LibraryBlock=on  DatabaseKey=788  SignalName=IN_DigitalOutputPWM.OUT_21_SENSE  SymbolName=IN_DigitalOutputPWM_OUT_21_SENSE_000788  DataType=uint16  Init=0  Slope=1  Bias=0  DataSize=1  fpDataType=uint16  BlockIOType=Inport  DeviceType=0
  in_IN_DigitalOutputPWM.OUT_21_SENSE_PULSE : KIBES_Signal/KIBES_Signal  MBDS_LibraryBlock=on  DatabaseKey=2222  SignalName=IN_DigitalOutputPWM.OUT_21_SENSE_PULSE  SymbolName=IN_DigitalOutputPWM_OUT_21_SENSE_PULSE_002222  DataType=uint16  Init=0  Slope=1  Bias=0  DataSize=1  fpDataType=uint16  BlockIOType=Inport  DeviceType=0
  in_IN_DigitalOutputPWM.OUT_21_TD : KIBES_Signal/KIBES_Signal  MBDS_LibraryBlock=on  DatabaseKey=791  SignalName=IN_DigitalOutputPWM.OUT_21_TD  SymbolName=IN_DigitalOutputPWM_OUT_21_TD_000791  DataType=boolean  Init=0  Slope=1  Bias=0  DataSize=1  fpDataType=boolean  BlockIOType=Inport  DeviceType=0
  in_IN_DigitalOutputPWM.OUT_22_SENSE : KIBES_Signal/KIBES_Signal  MBDS_LibraryBlock=on  DatabaseKey=768  SignalName=IN_DigitalOutputPWM.OUT_22_SENSE  SymbolName=IN_DigitalOutputPWM_OUT_22_SENSE_000768  DataType=uint16  Init=0  Slope=1  Bias=0  DataSize=1  fpDataType=uint16  BlockIOType=Inport  DeviceType=0
  in_IN_DigitalOutputPWM.OUT_23_SENSE : KIBES_Signal/KIBES_Signal  MBDS_LibraryBlock=on  DatabaseKey=771  SignalName=IN_DigitalOutputPWM.OUT_23_SENSE  SymbolName=IN_DigitalOutputPWM_OUT_23_SENSE_000771  DataType=uint16  Init=0  Slope=1  Bias=0  DataSize=1  fpDataType=uint16  BlockIOType=Inport  DeviceType=0
  in_IN_DigitalOutputPWM.OUT_24_SENSE : KIBES_Signal/KIBES_Signal  MBDS_LibraryBlock=on  DatabaseKey=774  SignalName=IN_DigitalOutputPWM.OUT_24_SENSE  SymbolName=IN_DigitalOutputPWM_OUT_24_SENSE_000774  DataType=uint16  Init=0  Slope=1  Bias=0  DataSize=1  fpDataType=uint16  BlockIOType=Inport  DeviceType=0
  in_IN_DigitalOutputPWM.OUT_25_SENSE : KIBES_Signal/KIBES_Signal  MBDS_LibraryBlock=on  DatabaseKey=777  SignalName=IN_DigitalOutputPWM.OUT_25_SENSE  SymbolName=IN_DigitalOutputPWM_OUT_25_SENSE_000777  DataType=uint16  Init=0  Slope=1  Bias=0  DataSize=1  fpDataType=uint16  BlockIOType=Inport  DeviceType=0
  in_IN_DigitalOutputPWM.OUT_26_SENSE : KIBES_Signal/KIBES_Signal  MBDS_LibraryBlock=on  DatabaseKey=795  SignalName=IN_DigitalOutputPWM.OUT_26_SENSE  SymbolName=IN_DigitalOutputPWM_OUT_26_SENSE_000795  DataType=uint16  Init=0  Slope=1  Bias=0  DataSize=1  fpDataType=uint16  BlockIOType=Inport  DeviceType=0
  in_IN_DigitalOutputPWM.OUT_27_SENSE : KIBES_Signal/KIBES_Signal  MBDS_LibraryBlock=on  DatabaseKey=798  SignalName=IN_DigitalOutputPWM.OUT_27_SENSE  SymbolName=IN_DigitalOutputPWM_OUT_27_SENSE_000798  DataType=uint16  Init=0  Slope=1  Bias=0  DataSize=1  fpDataType=uint16  BlockIOType=Inport  DeviceType=0
  in_IN_PCAN.Rx_Ctrl.Out_Ctrl.MessageState : KIBES_Signal/KIBES_Signal  MBDS_LibraryBlock=on  DatabaseKey=1715  SignalName=IN_PCAN.Rx_Ctrl.Out_Ctrl.MessageState  SymbolName=IN_PCAN_Rx_Ctrl_Out_Ctrl_MessageState_001715  DataType=uint16  Init=0  Slope=1  Bias=0  DataSize=1  fpDataType=uint16  BlockIOType=Inport  DeviceType=0
  in_IN_PCAN.Rx_Ctrl.Out_Ctrl.Out_18_PWM_Ctrl : KIBES_Signal/KIBES_Signal  MBDS_LibraryBlock=on  DatabaseKey=2295  SignalName=IN_PCAN.Rx_Ctrl.Out_Ctrl.Out_18_PWM_Ctrl  SymbolName=IN_PCAN_Rx_Ctrl_Out_Ctrl_Out_18_PWM_Ctrl_002295  DataType=uint8  Init=0  Slope=1  Bias=0  DataSize=1  fpDataType=uint8  BlockIOType=Inport  DeviceType=0
  in_IN_PCAN.Rx_Ctrl.Out_PWM_Ctrl.MessageState : KIBES_Signal/KIBES_Signal  MBDS_LibraryBlock=on  DatabaseKey=1717  SignalName=IN_PCAN.Rx_Ctrl.Out_PWM_Ctrl.MessageState  SymbolName=IN_PCAN_Rx_Ctrl_Out_PWM_Ctrl_MessageState_001717  DataType=uint16  Init=0  Slope=1  Bias=0  DataSize=1  fpDataType=uint16  BlockIOType=Inport  DeviceType=0
  in_IN_PCAN.Rx_Ctrl.Out_PWM_Ctrl.Out_20_PWM_Ctrl : KIBES_Signal/KIBES_Signal  MBDS_LibraryBlock=on  DatabaseKey=1711  SignalName=IN_PCAN.Rx_Ctrl.Out_PWM_Ctrl.Out_20_PWM_Ctrl  SymbolName=IN_PCAN_Rx_Ctrl_Out_PWM_Ctrl_Out_20_PWM_Ctrl_001711  DataType=uint8  Init=0  Slope=1  Bias=0  DataSize=1  fpDataType=uint8  BlockIOType=Inport  DeviceType=0
  in_IN_PCAN.Rx_Ctrl.Out_PWM_Ctrl.Out_21_PWM_Ctrl : KIBES_Signal/KIBES_Signal  MBDS_LibraryBlock=on  DatabaseKey=1710  SignalName=IN_PCAN.Rx_Ctrl.Out_PWM_Ctrl.Out_21_PWM_Ctrl  SymbolName=IN_PCAN_Rx_Ctrl_Out_PWM_Ctrl_Out_21_PWM_Ctrl_001710  DataType=uint8  Init=0  Slope=1  Bias=0  DataSize=1  fpDataType=uint8  BlockIOType=Inport  DeviceType=0
  in_IN_PCAN.Rx_Ctrl.Out_PWM_Ctrl.Out_22_PWM_Ctrl : KIBES_Signal/KIBES_Signal  MBDS_LibraryBlock=on  DatabaseKey=1709  SignalName=IN_PCAN.Rx_Ctrl.Out_PWM_Ctrl.Out_22_PWM_Ctrl  SymbolName=IN_PCAN_Rx_Ctrl_Out_PWM_Ctrl_Out_22_PWM_Ctrl_001709  DataType=uint8  Init=0  Slope=1  Bias=0  DataSize=1  fpDataType=uint8  BlockIOType=Inport  DeviceType=0
  in_IN_PCAN.Rx_Ctrl.Out_PWM_Ctrl.Out_23_PWM_Ctrl : KIBES_Signal/KIBES_Signal  MBDS_LibraryBlock=on  DatabaseKey=1708  SignalName=IN_PCAN.Rx_Ctrl.Out_PWM_Ctrl.Out_23_PWM_Ctrl  SymbolName=IN_PCAN_Rx_Ctrl_Out_PWM_Ctrl_Out_23_PWM_Ctrl_001708  DataType=uint8  Init=0  Slope=1  Bias=0  DataSize=1  fpDataType=uint8  BlockIOType=Inport  DeviceType=0
  in_IN_PCAN.Rx_Ctrl.Out_PWM_Ctrl.Out_24_PWM_Ctrl : KIBES_Signal/KIBES_Signal  MBDS_LibraryBlock=on  DatabaseKey=1707  SignalName=IN_PCAN.Rx_Ctrl.Out_PWM_Ctrl.Out_24_PWM_Ctrl  SymbolName=IN_PCAN_Rx_Ctrl_Out_PWM_Ctrl_Out_24_PWM_Ctrl_001707  DataType=uint8  Init=0  Slope=1  Bias=0  DataSize=1  fpDataType=uint8  BlockIOType=Inport  DeviceType=0
  in_IN_PCAN.Rx_Ctrl.Out_PWM_Ctrl.Out_25_PWM_Ctrl : KIBES_Signal/KIBES_Signal  MBDS_LibraryBlock=on  DatabaseKey=1706  SignalName=IN_PCAN.Rx_Ctrl.Out_PWM_Ctrl.Out_25_PWM_Ctrl  SymbolName=IN_PCAN_Rx_Ctrl_Out_PWM_Ctrl_Out_25_PWM_Ctrl_001706  DataType=uint8  Init=0  Slope=1  Bias=0  DataSize=1  fpDataType=uint8  BlockIOType=Inport  DeviceType=0
  in_IN_PCAN.Rx_Ctrl.Out_PWM_Ctrl.Out_26_PWM_Ctrl : KIBES_Signal/KIBES_Signal  MBDS_LibraryBlock=on  DatabaseKey=1705  SignalName=IN_PCAN.Rx_Ctrl.Out_PWM_Ctrl.Out_26_PWM_Ctrl  SymbolName=IN_PCAN_Rx_Ctrl_Out_PWM_Ctrl_Out_26_PWM_Ctrl_001705  DataType=uint8  Init=0  Slope=1  Bias=0  DataSize=1  fpDataType=uint8  BlockIOType=Inport  DeviceType=0
  in_IN_PCAN.Rx_Ctrl.Out_PWM_Ctrl.Out_27_PWM_Ctrl : KIBES_Signal/KIBES_Signal  MBDS_LibraryBlock=on  DatabaseKey=1704  SignalName=IN_PCAN.Rx_Ctrl.Out_PWM_Ctrl.Out_27_PWM_Ctrl  SymbolName=IN_PCAN_Rx_Ctrl_Out_PWM_Ctrl_Out_27_PWM_Ctrl_001704  DataType=uint8  Init=0  Slope=1  Bias=0  DataSize=1  fpDataType=uint8  BlockIOType=Inport  DeviceType=0
  out_OUT_DigitalOutputPWM.OUT_18_PWM : KIBES_Signal/KIBES_Signal  MBDS_LibraryBlock=on  DatabaseKey=2282  SignalName=OUT_DigitalOutputPWM.OUT_18_PWM  SymbolName=OUT_DigitalOutputPWM_OUT_18_PWM_002282  DataType=uint8  Init=0  Slope=1  Bias=0  DataSize=1  fpDataType=uint8  BlockIOType=Outport  DeviceType=0
  out_OUT_DigitalOutputPWM.OUT_20_PWM : KIBES_Signal/KIBES_Signal  MBDS_LibraryBlock=on  DatabaseKey=799  SignalName=OUT_DigitalOutputPWM.OUT_20_PWM  SymbolName=OUT_DigitalOutputPWM_OUT_20_PWM_000799  DataType=uint8  Init=0  Slope=1  Bias=0  DataSize=1  fpDataType=uint8  BlockIOType=Outport  DeviceType=0
  out_OUT_DigitalOutputPWM.OUT_20_TD_START : KIBES_Signal/KIBES_Signal  MBDS_LibraryBlock=on  DatabaseKey=785  SignalName=OUT_DigitalOutputPWM.OUT_20_TD_START  SymbolName=OUT_DigitalOutputPWM_OUT_20_TD_START_000785  DataType=boolean  Init=0  Slope=1  Bias=0  DataSize=1  fpDataType=boolean  BlockIOType=Outport  DeviceType=0
  out_OUT_DigitalOutputPWM.OUT_21_PWM : KIBES_Signal/KIBES_Signal  MBDS_LibraryBlock=on  DatabaseKey=786  SignalName=OUT_DigitalOutputPWM.OUT_21_PWM  SymbolName=OUT_DigitalOutputPWM_OUT_21_PWM_000786  DataType=uint8  Init=0  Slope=1  Bias=0  DataSize=1  fpDataType=uint8  BlockIOType=Outport  DeviceType=0
  out_OUT_DigitalOutputPWM.OUT_21_TD_START : KIBES_Signal/KIBES_Signal  MBDS_LibraryBlock=on  DatabaseKey=793  SignalName=OUT_DigitalOutputPWM.OUT_21_TD_START  SymbolName=OUT_DigitalOutputPWM_OUT_21_TD_START_000793  DataType=boolean  Init=0  Slope=1  Bias=0  DataSize=1  fpDataType=boolean  BlockIOType=Outport  DeviceType=0
  out_OUT_DigitalOutputPWM.OUT_22_PWM : KIBES_Signal/KIBES_Signal  MBDS_LibraryBlock=on  DatabaseKey=766  SignalName=OUT_DigitalOutputPWM.OUT_22_PWM  SymbolName=OUT_DigitalOutputPWM_OUT_22_PWM_000766  DataType=uint8  Init=0  Slope=1  Bias=0  DataSize=1  fpDataType=uint8  BlockIOType=Outport  DeviceType=0
  out_OUT_DigitalOutputPWM.OUT_23_PWM : KIBES_Signal/KIBES_Signal  MBDS_LibraryBlock=on  DatabaseKey=769  SignalName=OUT_DigitalOutputPWM.OUT_23_PWM  SymbolName=OUT_DigitalOutputPWM_OUT_23_PWM_000769  DataType=uint8  Init=0  Slope=1  Bias=0  DataSize=1  fpDataType=uint8  BlockIOType=Outport  DeviceType=0
  out_OUT_DigitalOutputPWM.OUT_24_PWM : KIBES_Signal/KIBES_Signal  MBDS_LibraryBlock=on  DatabaseKey=772  SignalName=OUT_DigitalOutputPWM.OUT_24_PWM  SymbolName=OUT_DigitalOutputPWM_OUT_24_PWM_000772  DataType=uint8  Init=0  Slope=1  Bias=0  DataSize=1  fpDataType=uint8  BlockIOType=Outport  DeviceType=0
  out_OUT_DigitalOutputPWM.OUT_25_PWM : KIBES_Signal/KIBES_Signal  MBDS_LibraryBlock=on  DatabaseKey=775  SignalName=OUT_DigitalOutputPWM.OUT_25_PWM  SymbolName=OUT_DigitalOutputPWM_OUT_25_PWM_000775  DataType=uint8  Init=0  Slope=1  Bias=0  DataSize=1  fpDataType=uint8  BlockIOType=Outport  DeviceType=0
  out_OUT_DigitalOutputPWM.OUT_26_PWM : KIBES_Signal/KIBES_Signal  MBDS_LibraryBlock=on  DatabaseKey=778  SignalName=OUT_DigitalOutputPWM.OUT_26_PWM  SymbolName=OUT_DigitalOutputPWM_OUT_26_PWM_000778  DataType=uint8  Init=0  Slope=1  Bias=0  DataSize=1  fpDataType=uint8  BlockIOType=Outport  DeviceType=0
  out_OUT_DigitalOutputPWM.OUT_27_PWM : KIBES_Signal/KIBES_Signal  MBDS_LibraryBlock=on  DatabaseKey=796  SignalName=OUT_DigitalOutputPWM.OUT_27_PWM  SymbolName=OUT_DigitalOutputPWM_OUT_27_PWM_000796  DataType=uint8  Init=0  Slope=1  Bias=0  DataSize=1  fpDataType=uint8  BlockIOType=Outport  DeviceType=0
  out_OUT_PCAN.Rx_Ctrl.Out_PWM_Ctrl.MessageEnable : KIBES_Signal/KIBES_Signal  MBDS_LibraryBlock=on  DatabaseKey=1716  SignalName=OUT_PCAN.Rx_Ctrl.Out_PWM_Ctrl.MessageEnable  SymbolName=OUT_PCAN_Rx_Ctrl_Out_PWM_Ctrl_MessageEnable_001716  DataType=boolean  Init=0  Slope=1  Bias=0  DataSize=1  fpDataType=boolean  BlockIOType=Outport  DeviceType=0
  out_OUT_PCAN.Tx_Out.Out_18_Sts.MessageEnable : KIBES_Signal/KIBES_Signal  MBDS_LibraryBlock=on  DatabaseKey=1666  SignalName=OUT_PCAN.Tx_Out.Out_18_Sts.MessageEnable  SymbolName=OUT_PCAN_Tx_Out_Out_18_Sts_MessageEnable_001666  DataType=boolean  Init=0  Slope=1  Bias=0  DataSize=1  fpDataType=boolean  BlockIOType=Outport  DeviceType=0
  out_OUT_PCAN.Tx_Out.Out_18_Sts.Out_DIAG : KIBES_Signal/KIBES_Signal  MBDS_LibraryBlock=on  DatabaseKey=1610  SignalName=OUT_PCAN.Tx_Out.Out_18_Sts.Out_DIAG  SymbolName=OUT_PCAN_Tx_Out_Out_18_Sts_Out_DIAG_001610  DataType=uint16  Init=0  Slope=1  Bias=0  DataSize=1  fpDataType=uint16  BlockIOType=Outport  DeviceType=0
  out_OUT_PCAN.Tx_Out.Out_18_Sts.Out_SENSE : KIBES_Signal/KIBES_Signal  MBDS_LibraryBlock=on  DatabaseKey=1609  SignalName=OUT_PCAN.Tx_Out.Out_18_Sts.Out_SENSE  SymbolName=OUT_PCAN_Tx_Out_Out_18_Sts_Out_SENSE_001609  DataType=uint16  Init=0  Slope=1  Bias=0  DataSize=1  fpDataType=uint16  BlockIOType=Outport  DeviceType=0
  out_OUT_PCAN.Tx_Out.Out_18_Sts.Out_STATUS : KIBES_Signal/KIBES_Signal  MBDS_LibraryBlock=on  DatabaseKey=1611  SignalName=OUT_PCAN.Tx_Out.Out_18_Sts.Out_STATUS  SymbolName=OUT_PCAN_Tx_Out_Out_18_Sts_Out_STATUS_001611  DataType=uint8  Init=0  Slope=1  Bias=0  DataSize=1  fpDataType=uint8  BlockIOType=Outport  DeviceType=0
  out_OUT_PCAN.Tx_Out.Out_20_Sts.MessageEnable : KIBES_Signal/KIBES_Signal  MBDS_LibraryBlock=on  DatabaseKey=1668  SignalName=OUT_PCAN.Tx_Out.Out_20_Sts.MessageEnable  SymbolName=OUT_PCAN_Tx_Out_Out_20_Sts_MessageEnable_001668  DataType=boolean  Init=0  Slope=1  Bias=0  DataSize=1  fpDataType=boolean  BlockIOType=Outport  DeviceType=0
  out_OUT_PCAN.Tx_Out.Out_20_Sts.Out_DIAG : KIBES_Signal/KIBES_Signal  MBDS_LibraryBlock=on  DatabaseKey=1618  SignalName=OUT_PCAN.Tx_Out.Out_20_Sts.Out_DIAG  SymbolName=OUT_PCAN_Tx_Out_Out_20_Sts_Out_DIAG_001618  DataType=uint16  Init=0  Slope=1  Bias=0  DataSize=1  fpDataType=uint16  BlockIOType=Outport  DeviceType=0
  out_OUT_PCAN.Tx_Out.Out_20_Sts.Out_SENSE : KIBES_Signal/KIBES_Signal  MBDS_LibraryBlock=on  DatabaseKey=1617  SignalName=OUT_PCAN.Tx_Out.Out_20_Sts.Out_SENSE  SymbolName=OUT_PCAN_Tx_Out_Out_20_Sts_Out_SENSE_001617  DataType=uint16  Init=0  Slope=1  Bias=0  DataSize=1  fpDataType=uint16  BlockIOType=Outport  DeviceType=0
  out_OUT_PCAN.Tx_Out.Out_20_Sts.Out_STATUS : KIBES_Signal/KIBES_Signal  MBDS_LibraryBlock=on  DatabaseKey=1619  SignalName=OUT_PCAN.Tx_Out.Out_20_Sts.Out_STATUS  SymbolName=OUT_PCAN_Tx_Out_Out_20_Sts_Out_STATUS_001619  DataType=uint8  Init=0  Slope=1  Bias=0  DataSize=1  fpDataType=uint8  BlockIOType=Outport  DeviceType=0
  out_OUT_PCAN.Tx_Out.Out_20_Sts.Out_TD : KIBES_Signal/KIBES_Signal  MBDS_LibraryBlock=on  DatabaseKey=1616  SignalName=OUT_PCAN.Tx_Out.Out_20_Sts.Out_TD  SymbolName=OUT_PCAN_Tx_Out_Out_20_Sts_Out_TD_001616  DataType=boolean  Init=0  Slope=1  Bias=0  DataSize=1  fpDataType=boolean  BlockIOType=Outport  DeviceType=0
  out_OUT_PCAN.Tx_Out.Out_20_Sts.Out_TD_DIAG : KIBES_Signal/KIBES_Signal  MBDS_LibraryBlock=on  DatabaseKey=1615  SignalName=OUT_PCAN.Tx_Out.Out_20_Sts.Out_TD_DIAG  SymbolName=OUT_PCAN_Tx_Out_Out_20_Sts_Out_TD_DIAG_001615  DataType=uint16  Init=0  Slope=1  Bias=0  DataSize=1  fpDataType=uint16  BlockIOType=Outport  DeviceType=0
  out_OUT_PCAN.Tx_Out.Out_20_TD_Sts.MessageEnable : KIBES_Signal/KIBES_Signal  MBDS_LibraryBlock=on  DatabaseKey=2200  SignalName=OUT_PCAN.Tx_Out.Out_20_TD_Sts.MessageEnable  SymbolName=OUT_PCAN_Tx_Out_Out_20_TD_Sts_MessageEnable_002200  DataType=boolean  Init=0  Slope=1  Bias=0  DataSize=1  fpDataType=boolean  BlockIOType=Outport  DeviceType=0
  out_OUT_PCAN.Tx_Out.Out_20_TD_Sts.Out_SENSE_PULSE : KIBES_Signal/KIBES_Signal  MBDS_LibraryBlock=on  DatabaseKey=2187  SignalName=OUT_PCAN.Tx_Out.Out_20_TD_Sts.Out_SENSE_PULSE  SymbolName=OUT_PCAN_Tx_Out_Out_20_TD_Sts_Out_SENSE_PULSE_002187  DataType=uint16  Init=0  Slope=1  Bias=0  DataSize=1  fpDataType=uint16  BlockIOType=Outport  DeviceType=0
  out_OUT_PCAN.Tx_Out.Out_20_TD_Sts.Out_SENSE_PULSE_DIAG : KIBES_Signal/KIBES_Signal  MBDS_LibraryBlock=on  DatabaseKey=2188  SignalName=OUT_PCAN.Tx_Out.Out_20_TD_Sts.Out_SENSE_PULSE_DIAG  SymbolName=OUT_PCAN_Tx_Out_Out_20_TD_Sts_Out_SENSE_PULSE_DIAG_002188  DataType=uint16  Init=0  Slope=1  Bias=0  DataSize=1  fpDataType=uint16  BlockIOType=Outport  DeviceType=0
  out_OUT_PCAN.Tx_Out.Out_21_Sts.MessageEnable : KIBES_Signal/KIBES_Signal  MBDS_LibraryBlock=on  DatabaseKey=1669  SignalName=OUT_PCAN.Tx_Out.Out_21_Sts.MessageEnable  SymbolName=OUT_PCAN_Tx_Out_Out_21_Sts_MessageEnable_001669  DataType=boolean  Init=0  Slope=1  Bias=0  DataSize=1  fpDataType=boolean  BlockIOType=Outport  DeviceType=0
  out_OUT_PCAN.Tx_Out.Out_21_Sts.Out_DIAG : KIBES_Signal/KIBES_Signal  MBDS_LibraryBlock=on  DatabaseKey=1623  SignalName=OUT_PCAN.Tx_Out.Out_21_Sts.Out_DIAG  SymbolName=OUT_PCAN_Tx_Out_Out_21_Sts_Out_DIAG_001623  DataType=uint16  Init=0  Slope=1  Bias=0  DataSize=1  fpDataType=uint16  BlockIOType=Outport  DeviceType=0
  out_OUT_PCAN.Tx_Out.Out_21_Sts.Out_SENSE : KIBES_Signal/KIBES_Signal  MBDS_LibraryBlock=on  DatabaseKey=1622  SignalName=OUT_PCAN.Tx_Out.Out_21_Sts.Out_SENSE  SymbolName=OUT_PCAN_Tx_Out_Out_21_Sts_Out_SENSE_001622  DataType=uint16  Init=0  Slope=1  Bias=0  DataSize=1  fpDataType=uint16  BlockIOType=Outport  DeviceType=0
  out_OUT_PCAN.Tx_Out.Out_21_Sts.Out_STATUS : KIBES_Signal/KIBES_Signal  MBDS_LibraryBlock=on  DatabaseKey=1624  SignalName=OUT_PCAN.Tx_Out.Out_21_Sts.Out_STATUS  SymbolName=OUT_PCAN_Tx_Out_Out_21_Sts_Out_STATUS_001624  DataType=uint8  Init=0  Slope=1  Bias=0  DataSize=1  fpDataType=uint8  BlockIOType=Outport  DeviceType=0
  out_OUT_PCAN.Tx_Out.Out_21_Sts.Out_TD : KIBES_Signal/KIBES_Signal  MBDS_LibraryBlock=on  DatabaseKey=1621  SignalName=OUT_PCAN.Tx_Out.Out_21_Sts.Out_TD  SymbolName=OUT_PCAN_Tx_Out_Out_21_Sts_Out_TD_001621  DataType=boolean  Init=0  Slope=1  Bias=0  DataSize=1  fpDataType=boolean  BlockIOType=Outport  DeviceType=0
  out_OUT_PCAN.Tx_Out.Out_21_Sts.Out_TD_DIAG : KIBES_Signal/KIBES_Signal  MBDS_LibraryBlock=on  DatabaseKey=1620  SignalName=OUT_PCAN.Tx_Out.Out_21_Sts.Out_TD_DIAG  SymbolName=OUT_PCAN_Tx_Out_Out_21_Sts_Out_TD_DIAG_001620  DataType=uint16  Init=0  Slope=1  Bias=0  DataSize=1  fpDataType=uint16  BlockIOType=Outport  DeviceType=0
  out_OUT_PCAN.Tx_Out.Out_21_TD_Sts.MessageEnable : KIBES_Signal/KIBES_Signal  MBDS_LibraryBlock=on  DatabaseKey=2201  SignalName=OUT_PCAN.Tx_Out.Out_21_TD_Sts.MessageEnable  SymbolName=OUT_PCAN_Tx_Out_Out_21_TD_Sts_MessageEnable_002201  DataType=boolean  Init=0  Slope=1  Bias=0  DataSize=1  fpDataType=boolean  BlockIOType=Outport  DeviceType=0
  out_OUT_PCAN.Tx_Out.Out_21_TD_Sts.Out_SENSE_PULSE : KIBES_Signal/KIBES_Signal  MBDS_LibraryBlock=on  DatabaseKey=2189  SignalName=OUT_PCAN.Tx_Out.Out_21_TD_Sts.Out_SENSE_PULSE  SymbolName=OUT_PCAN_Tx_Out_Out_21_TD_Sts_Out_SENSE_PULSE_002189  DataType=uint16  Init=0  Slope=1  Bias=0  DataSize=1  fpDataType=uint16  BlockIOType=Outport  DeviceType=0
  out_OUT_PCAN.Tx_Out.Out_21_TD_Sts.Out_SENSE_PULSE_DIAG : KIBES_Signal/KIBES_Signal  MBDS_LibraryBlock=on  DatabaseKey=2190  SignalName=OUT_PCAN.Tx_Out.Out_21_TD_Sts.Out_SENSE_PULSE_DIAG  SymbolName=OUT_PCAN_Tx_Out_Out_21_TD_Sts_Out_SENSE_PULSE_DIAG_002190  DataType=uint16  Init=0  Slope=1  Bias=0  DataSize=1  fpDataType=uint16  BlockIOType=Outport  DeviceType=0
  out_OUT_PCAN.Tx_Out.Out_22_Sts.MessageEnable : KIBES_Signal/KIBES_Signal  MBDS_LibraryBlock=on  DatabaseKey=1670  SignalName=OUT_PCAN.Tx_Out.Out_22_Sts.MessageEnable  SymbolName=OUT_PCAN_Tx_Out_Out_22_Sts_MessageEnable_001670  DataType=boolean  Init=0  Slope=1  Bias=0  DataSize=1  fpDataType=boolean  BlockIOType=Outport  DeviceType=0
  out_OUT_PCAN.Tx_Out.Out_22_Sts.Out_DIAG : KIBES_Signal/KIBES_Signal  MBDS_LibraryBlock=on  DatabaseKey=1626  SignalName=OUT_PCAN.Tx_Out.Out_22_Sts.Out_DIAG  SymbolName=OUT_PCAN_Tx_Out_Out_22_Sts_Out_DIAG_001626  DataType=uint16  Init=0  Slope=1  Bias=0  DataSize=1  fpDataType=uint16  BlockIOType=Outport  DeviceType=0
  out_OUT_PCAN.Tx_Out.Out_22_Sts.Out_SENSE : KIBES_Signal/KIBES_Signal  MBDS_LibraryBlock=on  DatabaseKey=1625  SignalName=OUT_PCAN.Tx_Out.Out_22_Sts.Out_SENSE  SymbolName=OUT_PCAN_Tx_Out_Out_22_Sts_Out_SENSE_001625  DataType=uint16  Init=0  Slope=1  Bias=0  DataSize=1  fpDataType=uint16  BlockIOType=Outport  DeviceType=0
  out_OUT_PCAN.Tx_Out.Out_22_Sts.Out_STATUS : KIBES_Signal/KIBES_Signal  MBDS_LibraryBlock=on  DatabaseKey=1627  SignalName=OUT_PCAN.Tx_Out.Out_22_Sts.Out_STATUS  SymbolName=OUT_PCAN_Tx_Out_Out_22_Sts_Out_STATUS_001627  DataType=uint8  Init=0  Slope=1  Bias=0  DataSize=1  fpDataType=uint8  BlockIOType=Outport  DeviceType=0
  out_OUT_PCAN.Tx_Out.Out_23_Sts.MessageEnable : KIBES_Signal/KIBES_Signal  MBDS_LibraryBlock=on  DatabaseKey=1671  SignalName=OUT_PCAN.Tx_Out.Out_23_Sts.MessageEnable  SymbolName=OUT_PCAN_Tx_Out_Out_23_Sts_MessageEnable_001671  DataType=boolean  Init=0  Slope=1  Bias=0  DataSize=1  fpDataType=boolean  BlockIOType=Outport  DeviceType=0
  out_OUT_PCAN.Tx_Out.Out_23_Sts.Out_DIAG : KIBES_Signal/KIBES_Signal  MBDS_LibraryBlock=on  DatabaseKey=1629  SignalName=OUT_PCAN.Tx_Out.Out_23_Sts.Out_DIAG  SymbolName=OUT_PCAN_Tx_Out_Out_23_Sts_Out_DIAG_001629  DataType=uint16  Init=0  Slope=1  Bias=0  DataSize=1  fpDataType=uint16  BlockIOType=Outport  DeviceType=0
  out_OUT_PCAN.Tx_Out.Out_23_Sts.Out_SENSE : KIBES_Signal/KIBES_Signal  MBDS_LibraryBlock=on  DatabaseKey=1628  SignalName=OUT_PCAN.Tx_Out.Out_23_Sts.Out_SENSE  SymbolName=OUT_PCAN_Tx_Out_Out_23_Sts_Out_SENSE_001628  DataType=uint16  Init=0  Slope=1  Bias=0  DataSize=1  fpDataType=uint16  BlockIOType=Outport  DeviceType=0
  out_OUT_PCAN.Tx_Out.Out_23_Sts.Out_STATUS : KIBES_Signal/KIBES_Signal  MBDS_LibraryBlock=on  DatabaseKey=1630  SignalName=OUT_PCAN.Tx_Out.Out_23_Sts.Out_STATUS  SymbolName=OUT_PCAN_Tx_Out_Out_23_Sts_Out_STATUS_001630  DataType=uint8  Init=0  Slope=1  Bias=0  DataSize=1  fpDataType=uint8  BlockIOType=Outport  DeviceType=0
  out_OUT_PCAN.Tx_Out.Out_24_Sts.MessageEnable : KIBES_Signal/KIBES_Signal  MBDS_LibraryBlock=on  DatabaseKey=1672  SignalName=OUT_PCAN.Tx_Out.Out_24_Sts.MessageEnable  SymbolName=OUT_PCAN_Tx_Out_Out_24_Sts_MessageEnable_001672  DataType=boolean  Init=0  Slope=1  Bias=0  DataSize=1  fpDataType=boolean  BlockIOType=Outport  DeviceType=0
  out_OUT_PCAN.Tx_Out.Out_24_Sts.Out_DIAG : KIBES_Signal/KIBES_Signal  MBDS_LibraryBlock=on  DatabaseKey=1632  SignalName=OUT_PCAN.Tx_Out.Out_24_Sts.Out_DIAG  SymbolName=OUT_PCAN_Tx_Out_Out_24_Sts_Out_DIAG_001632  DataType=uint16  Init=0  Slope=1  Bias=0  DataSize=1  fpDataType=uint16  BlockIOType=Outport  DeviceType=0
  out_OUT_PCAN.Tx_Out.Out_24_Sts.Out_SENSE : KIBES_Signal/KIBES_Signal  MBDS_LibraryBlock=on  DatabaseKey=1631  SignalName=OUT_PCAN.Tx_Out.Out_24_Sts.Out_SENSE  SymbolName=OUT_PCAN_Tx_Out_Out_24_Sts_Out_SENSE_001631  DataType=uint16  Init=0  Slope=1  Bias=0  DataSize=1  fpDataType=uint16  BlockIOType=Outport  DeviceType=0
  out_OUT_PCAN.Tx_Out.Out_24_Sts.Out_STATUS : KIBES_Signal/KIBES_Signal  MBDS_LibraryBlock=on  DatabaseKey=1633  SignalName=OUT_PCAN.Tx_Out.Out_24_Sts.Out_STATUS  SymbolName=OUT_PCAN_Tx_Out_Out_24_Sts_Out_STATUS_001633  DataType=uint8  Init=0  Slope=1  Bias=0  DataSize=1  fpDataType=uint8  BlockIOType=Outport  DeviceType=0
  out_OUT_PCAN.Tx_Out.Out_25_Sts.MessageEnable : KIBES_Signal/KIBES_Signal  MBDS_LibraryBlock=on  DatabaseKey=1673  SignalName=OUT_PCAN.Tx_Out.Out_25_Sts.MessageEnable  SymbolName=OUT_PCAN_Tx_Out_Out_25_Sts_MessageEnable_001673  DataType=boolean  Init=0  Slope=1  Bias=0  DataSize=1  fpDataType=boolean  BlockIOType=Outport  DeviceType=0
  out_OUT_PCAN.Tx_Out.Out_25_Sts.Out_DIAG : KIBES_Signal/KIBES_Signal  MBDS_LibraryBlock=on  DatabaseKey=1635  SignalName=OUT_PCAN.Tx_Out.Out_25_Sts.Out_DIAG  SymbolName=OUT_PCAN_Tx_Out_Out_25_Sts_Out_DIAG_001635  DataType=uint16  Init=0  Slope=1  Bias=0  DataSize=1  fpDataType=uint16  BlockIOType=Outport  DeviceType=0
  out_OUT_PCAN.Tx_Out.Out_25_Sts.Out_SENSE : KIBES_Signal/KIBES_Signal  MBDS_LibraryBlock=on  DatabaseKey=1634  SignalName=OUT_PCAN.Tx_Out.Out_25_Sts.Out_SENSE  SymbolName=OUT_PCAN_Tx_Out_Out_25_Sts_Out_SENSE_001634  DataType=uint16  Init=0  Slope=1  Bias=0  DataSize=1  fpDataType=uint16  BlockIOType=Outport  DeviceType=0
  out_OUT_PCAN.Tx_Out.Out_25_Sts.Out_STATUS : KIBES_Signal/KIBES_Signal  MBDS_LibraryBlock=on  DatabaseKey=1636  SignalName=OUT_PCAN.Tx_Out.Out_25_Sts.Out_STATUS  SymbolName=OUT_PCAN_Tx_Out_Out_25_Sts_Out_STATUS_001636  DataType=uint8  Init=0  Slope=1  Bias=0  DataSize=1  fpDataType=uint8  BlockIOType=Outport  DeviceType=0
  out_OUT_PCAN.Tx_Out.Out_26_Sts.MessageEnable : KIBES_Signal/KIBES_Signal  MBDS_LibraryBlock=on  DatabaseKey=1674  SignalName=OUT_PCAN.Tx_Out.Out_26_Sts.MessageEnable  SymbolName=OUT_PCAN_Tx_Out_Out_26_Sts_MessageEnable_001674  DataType=boolean  Init=0  Slope=1  Bias=0  DataSize=1  fpDataType=boolean  BlockIOType=Outport  DeviceType=0
  out_OUT_PCAN.Tx_Out.Out_26_Sts.Out_DIAG : KIBES_Signal/KIBES_Signal  MBDS_LibraryBlock=on  DatabaseKey=1638  SignalName=OUT_PCAN.Tx_Out.Out_26_Sts.Out_DIAG  SymbolName=OUT_PCAN_Tx_Out_Out_26_Sts_Out_DIAG_001638  DataType=uint16  Init=0  Slope=1  Bias=0  DataSize=1  fpDataType=uint16  BlockIOType=Outport  DeviceType=0
  out_OUT_PCAN.Tx_Out.Out_26_Sts.Out_SENSE : KIBES_Signal/KIBES_Signal  MBDS_LibraryBlock=on  DatabaseKey=1637  SignalName=OUT_PCAN.Tx_Out.Out_26_Sts.Out_SENSE  SymbolName=OUT_PCAN_Tx_Out_Out_26_Sts_Out_SENSE_001637  DataType=uint16  Init=0  Slope=1  Bias=0  DataSize=1  fpDataType=uint16  BlockIOType=Outport  DeviceType=0
  out_OUT_PCAN.Tx_Out.Out_26_Sts.Out_STATUS : KIBES_Signal/KIBES_Signal  MBDS_LibraryBlock=on  DatabaseKey=1639  SignalName=OUT_PCAN.Tx_Out.Out_26_Sts.Out_STATUS  SymbolName=OUT_PCAN_Tx_Out_Out_26_Sts_Out_STATUS_001639  DataType=uint8  Init=0  Slope=1  Bias=0  DataSize=1  fpDataType=uint8  BlockIOType=Outport  DeviceType=0
  out_OUT_PCAN.Tx_Out.Out_27_Sts.MessageEnable : KIBES_Signal/KIBES_Signal  MBDS_LibraryBlock=on  DatabaseKey=1675  SignalName=OUT_PCAN.Tx_Out.Out_27_Sts.MessageEnable  SymbolName=OUT_PCAN_Tx_Out_Out_27_Sts_MessageEnable_001675  DataType=boolean  Init=0  Slope=1  Bias=0  DataSize=1  fpDataType=boolean  BlockIOType=Outport  DeviceType=0
  out_OUT_PCAN.Tx_Out.Out_27_Sts.Out_DIAG : KIBES_Signal/KIBES_Signal  MBDS_LibraryBlock=on  DatabaseKey=1641  SignalName=OUT_PCAN.Tx_Out.Out_27_Sts.Out_DIAG  SymbolName=OUT_PCAN_Tx_Out_Out_27_Sts_Out_DIAG_001641  DataType=uint16  Init=0  Slope=1  Bias=0  DataSize=1  fpDataType=uint16  BlockIOType=Outport  DeviceType=0
  out_OUT_PCAN.Tx_Out.Out_27_Sts.Out_SENSE : KIBES_Signal/KIBES_Signal  MBDS_LibraryBlock=on  DatabaseKey=1640  SignalName=OUT_PCAN.Tx_Out.Out_27_Sts.Out_SENSE  SymbolName=OUT_PCAN_Tx_Out_Out_27_Sts_Out_SENSE_001640  DataType=uint16  Init=0  Slope=1  Bias=0  DataSize=1  fpDataType=uint16  BlockIOType=Outport  DeviceType=0
  out_OUT_PCAN.Tx_Out.Out_27_Sts.Out_STATUS : KIBES_Signal/KIBES_Signal  MBDS_LibraryBlock=on  DatabaseKey=1642  SignalName=OUT_PCAN.Tx_Out.Out_27_Sts.Out_STATUS  SymbolName=OUT_PCAN_Tx_Out_Out_27_Sts_Out_STATUS_001642  DataType=uint8  Init=0  Slope=1  Bias=0  DataSize=1  fpDataType=uint8  BlockIOType=Outport  DeviceType=0
  wires:
  in_DIAG_DigitalOutputPWM.OUT_21_TD_DIAG/1 -> out_OUT_PCAN.Tx_Out.Out_21_Sts.Out_TD_DIAG/1, [boOut21TDDiag]
  in_DIAG_DigitalOutputPWM.OUT_20_PWM_DIAG/1 -> [boOut20Diag], out_OUT_PCAN.Tx_Out.Out_20_Sts.Out_DIAG/1
  in_DIAG_DigitalOutputPWM.OUT_25_PWM_DIAG/1 -> [boOut25Diag], out_OUT_PCAN.Tx_Out.Out_25_Sts.Out_DIAG/1
  in_DIAG_DigitalOutputPWM.OUT_20_TD_DIAG/1 -> out_OUT_PCAN.Tx_Out.Out_20_Sts.Out_TD_DIAG/1, [boOut20TDDiag]
  in_DIAG_DigitalOutputPWM.OUT_23_PWM_DIAG/1 -> [boOut23Diag], out_OUT_PCAN.Tx_Out.Out_23_Sts.Out_DIAG/1
  in_DIAG_DigitalOutputPWM.OUT_24_PWM_DIAG/1 -> [boOut24Diag], out_OUT_PCAN.Tx_Out.Out_24_Sts.Out_DIAG/1
  in_DIAG_DigitalOutputPWM.OUT_21_PWM_DIAG/1 -> [boOut21Diag], out_OUT_PCAN.Tx_Out.Out_21_Sts.Out_DIAG/1
  in_DIAG_DigitalOutputPWM.OUT_22_PWM_DIAG/1 -> [boOut22Diag], out_OUT_PCAN.Tx_Out.Out_22_Sts.Out_DIAG/1
  in_DIAG_DigitalOutputPWM.OUT_26_PWM_DIAG/1 -> [boOut26Diag], out_OUT_PCAN.Tx_Out.Out_26_Sts.Out_DIAG/1
  in_DIAG_DigitalOutputPWM.OUT_27_PWM_DIAG/1 -> [boOut27Diag], out_OUT_PCAN.Tx_Out.Out_27_Sts.Out_DIAG/1
  bo_SendEnable/1 -> out_OUT_PCAN.Tx_Out.Out_27_Sts.MessageEnable/1, out_OUT_PCAN.Tx_Out.Out_26_Sts.MessageEnable/1, out_OUT_PCAN.Tx_Out.Out_25_Sts.MessageEnable/1, out_OUT_PCAN.Tx_Out.Out_24_Sts.MessageEnable/1, out_OUT_PCAN.Tx_Out.Out_23_Sts.MessageEnable/1, out_OUT_PCAN.Tx_Out.Out_22_Sts.MessageEnable/1, out_OUT_PCAN.Tx_Out.Out_21_TD_Sts.MessageEnable/1, out_OUT_PCAN.Tx_Out.Out_21_Sts.MessageEnable/1, out_OUT_PCAN.Tx_Out.Out_20_TD_Sts.MessageEnable/1, out_OUT_PCAN.Tx_Out.Out_20_Sts.MessageEnable/1, out_OUT_PCAN.Tx_Out.Out_18_Sts.MessageEnable/1
  in_IN_DigitalOutputPWM.OUT_20_SENSE/1 -> out_OUT_PCAN.Tx_Out.Out_20_Sts.Out_SENSE/1
  in_IN_DigitalOutputPWM.OUT_20_TD/1 -> out_OUT_PCAN.Tx_Out.Out_20_Sts.Out_TD/1, [boOut20TD]
  in_IN_DigitalOutputPWM.OUT_21_SENSE/1 -> out_OUT_PCAN.Tx_Out.Out_21_Sts.Out_SENSE/1
  in_IN_DigitalOutputPWM.OUT_21_TD/1 -> out_OUT_PCAN.Tx_Out.Out_21_Sts.Out_TD/1, [boOut21TD]
  in_IN_DigitalOutputPWM.OUT_22_SENSE/1 -> out_OUT_PCAN.Tx_Out.Out_22_Sts.Out_SENSE/1
  in_IN_DigitalOutputPWM.OUT_23_SENSE/1 -> out_OUT_PCAN.Tx_Out.Out_23_Sts.Out_SENSE/1
  in_IN_DigitalOutputPWM.OUT_24_SENSE/1 -> out_OUT_PCAN.Tx_Out.Out_24_Sts.Out_SENSE/1
  in_IN_DigitalOutputPWM.OUT_25_SENSE/1 -> out_OUT_PCAN.Tx_Out.Out_25_Sts.Out_SENSE/1
  in_IN_DigitalOutputPWM.OUT_26_SENSE/1 -> out_OUT_PCAN.Tx_Out.Out_26_Sts.Out_SENSE/1
  in_IN_DigitalOutputPWM.OUT_27_SENSE/1 -> out_OUT_PCAN.Tx_Out.Out_27_Sts.Out_SENSE/1
  EQ/1(y) -> [boCtrlValid]
  in_IN_PCAN.Rx_Ctrl.Out_PWM_Ctrl.MessageState/1 -> EQ/1(u1)
  Constant1/1 -> EQ1/2(u2), EQ/2(u2)
  MOD_OutputDiag_Ctrl_22/1 -> Switch2/2
  Constant2/1 -> Switch8/3, Switch7/3, Switch6/3, Switch5/3, Switch4/3, Switch3/3, Switch2/3
  [u8Out21Ctrl] -> Switch1/1
  in_IN_PCAN.Rx_Ctrl.Out_PWM_Ctrl.Out_22_PWM_Ctrl/1 -> GT3/1(u1), Switch2/1
  in_IN_PCAN.Rx_Ctrl.Out_PWM_Ctrl.Out_23_PWM_Ctrl/1 -> GT4/1(u1), Switch3/1
  in_IN_PCAN.Rx_Ctrl.Out_PWM_Ctrl.Out_24_PWM_Ctrl/1 -> Switch4/1, GT5/1(u1)
  in_IN_PCAN.Rx_Ctrl.Out_PWM_Ctrl.Out_25_PWM_Ctrl/1 -> GT6/1(u1), Switch5/1
  in_IN_PCAN.Rx_Ctrl.Out_PWM_Ctrl.Out_26_PWM_Ctrl/1 -> GT7/1(u1), Switch6/1
  in_IN_PCAN.Rx_Ctrl.Out_PWM_Ctrl.Out_27_PWM_Ctrl/1 -> GT8/1(u1), Switch7/1
  Constant3/1 -> out_OUT_PCAN.Rx_Ctrl.Out_PWM_Ctrl.MessageEnable/1
  Switch2/1 -> out_OUT_PCAN.Tx_Out.Out_22_Sts.Out_STATUS/1, out_OUT_DigitalOutputPWM.OUT_22_PWM/1
  Switch3/1 -> out_OUT_PCAN.Tx_Out.Out_23_Sts.Out_STATUS/1, out_OUT_DigitalOutputPWM.OUT_23_PWM/1
  Switch4/1 -> out_OUT_PCAN.Tx_Out.Out_24_Sts.Out_STATUS/1, out_OUT_DigitalOutputPWM.OUT_24_PWM/1
  Switch5/1 -> out_OUT_PCAN.Tx_Out.Out_25_Sts.Out_STATUS/1, out_OUT_DigitalOutputPWM.OUT_25_PWM/1
  Switch6/1 -> out_OUT_PCAN.Tx_Out.Out_26_Sts.Out_STATUS/1, out_OUT_DigitalOutputPWM.OUT_26_PWM/1
  Switch7/1 -> out_OUT_PCAN.Tx_Out.Out_27_Sts.Out_STATUS/1, out_OUT_DigitalOutputPWM.OUT_27_PWM/1
  [boOut20TD] -> MOD_TrailerDetection_Ctrl_20/2
  [boOut20TDDiag] -> MOD_TrailerDetection_Ctrl_20/3
  Constant4/1 -> [u8TdTimeout]
  [u8TdTimeout] -> MOD_TrailerDetection_Ctrl_20/4
  MOD_TrailerDetection_Ctrl_20/2 -> out_OUT_DigitalOutputPWM.OUT_20_TD_START/1
  [boOut20Rqst] -> MOD_TrailerDetection_Ctrl_20/1
  MOD_OutputDiag_Ctrl_21/1 -> Switch1/2
  Constant6/1 -> Switch1/3
  [u8TdTimeout] -> MOD_TrailerDetection_Ctrl_21/4
  [boOut21TDDiag] -> MOD_TrailerDetection_Ctrl_21/3
  [boOut21TD] -> MOD_TrailerDetection_Ctrl_21/2
  [boOut21Rqst] -> MOD_TrailerDetection_Ctrl_21/1
  Switch1/1 -> out_OUT_DigitalOutputPWM.OUT_21_PWM/1
  MOD_TrailerDetection_Ctrl_21/2 -> out_OUT_DigitalOutputPWM.OUT_21_TD_START/1
  [u8Out20Ctrl] -> Switch9/1
  Constant7/1 -> Switch9/3
  MOD_OutputDiag_Ctrl_20/1 -> Switch9/2
  Switch9/1 -> out_OUT_DigitalOutputPWM.OUT_20_PWM/1
  MOD_TrailerDetection_Ctrl_20/1 -> Data Type Conversion/1, [boOut20]
  in_IN_PCAN.Rx_Ctrl.Out_PWM_Ctrl.Out_20_PWM_Ctrl/1 -> [u8Out20Ctrl], GT/1(u1)
  Constant5/1 -> GT/2(u2)
  GT/1(y) -> AND/1(u1)
  [boCtrlValid] -> AND/2(u2)
  AND/1(y) -> [boOut20Rqst]
  Constant8/1 -> GT1/2(u2)
  AND1/1(y) -> [boOut21Rqst]
  in_IN_PCAN.Rx_Ctrl.Out_PWM_Ctrl.Out_21_PWM_Ctrl/1 -> [u8Out21Ctrl], GT1/1(u1)
  GT1/1(y) -> AND1/1(u1)
  [boCtrlValid] -> AND1/2(u2)
  MOD_TrailerDetection_Ctrl_21/1 -> Data Type Conversion1/1, [boOut21]
  Data Type Conversion/1 -> out_OUT_PCAN.Tx_Out.Out_20_Sts.Out_STATUS/1
  Data Type Conversion1/1 -> out_OUT_PCAN.Tx_Out.Out_21_Sts.Out_STATUS/1
  in_DIAG_DigitalOutputPWM.OUT_20_SENSE_PULSE_DIAG/1 -> out_OUT_PCAN.Tx_Out.Out_20_TD_Sts.Out_SENSE_PULSE_DIAG/1
  in_IN_DigitalOutputPWM.OUT_20_SENSE_PULSE/1 -> out_OUT_PCAN.Tx_Out.Out_20_TD_Sts.Out_SENSE_PULSE/1
  in_IN_DigitalOutputPWM.OUT_21_SENSE_PULSE/1 -> out_OUT_PCAN.Tx_Out.Out_21_TD_Sts.Out_SENSE_PULSE/1
  in_DIAG_DigitalOutputPWM.OUT_21_SENSE_PULSE_DIAG/1 -> out_OUT_PCAN.Tx_Out.Out_21_TD_Sts.Out_SENSE_PULSE_DIAG/1
  Switch8/1 -> out_OUT_PCAN.Tx_Out.Out_18_Sts.Out_STATUS/1, out_OUT_DigitalOutputPWM.OUT_18_PWM/1
  in_DIAG_DigitalOutputPWM.OUT_18_PWM_DIAG/1 -> [boOut18Diag], out_OUT_PCAN.Tx_Out.Out_18_Sts.Out_DIAG/1
  in_IN_DigitalOutputPWM.OUT_18_SENSE/1 -> out_OUT_PCAN.Tx_Out.Out_18_Sts.Out_SENSE/1
  in_IN_PCAN.Rx_Ctrl.Out_Ctrl.Out_18_PWM_Ctrl/1 -> GT2/1(u1), Switch8/1
  [boOut20] -> MOD_OutputDiag_Ctrl_20/1
  in_IN_PCAN.Rx_Ctrl.Out_Ctrl.MessageState/1 -> EQ1/1(u1)
  EQ1/1(y) -> [boCtrl18Valid]
  MOD_OutputDiag_Ctrl_18/1 -> Switch8/2
  [boOut20Diag] -> MOD_OutputDiag_Ctrl_20/2
  [boCtrlValid] -> MOD_OutputDiag_Ctrl_20/3
  [boOut21] -> MOD_OutputDiag_Ctrl_21/1
  [boOut21Diag] -> MOD_OutputDiag_Ctrl_21/2
  [boCtrlValid] -> MOD_OutputDiag_Ctrl_21/3
  [boCtrl18Valid] -> MOD_OutputDiag_Ctrl_18/3
  Constant9/1 -> GT2/2(u2)
  GT2/1(y) -> MOD_OutputDiag_Ctrl_18/1
  [boOut18Diag] -> MOD_OutputDiag_Ctrl_18/2
  [boCtrlValid] -> MOD_OutputDiag_Ctrl_22/3
  GT3/1(y) -> MOD_OutputDiag_Ctrl_22/1
  Constant10/1 -> GT3/2(u2)
  [boOut22Diag] -> MOD_OutputDiag_Ctrl_22/2
  Constant11/1 -> GT4/2(u2)
  [boOut23Diag] -> MOD_OutputDiag_Ctrl_23/2
  GT4/1(y) -> MOD_OutputDiag_Ctrl_23/1
  [boCtrlValid] -> MOD_OutputDiag_Ctrl_23/3
  MOD_OutputDiag_Ctrl_23/1 -> Switch3/2
  Constant12/1 -> GT5/2(u2)
  [boCtrlValid] -> MOD_OutputDiag_Ctrl_24/3
  [boOut24Diag] -> MOD_OutputDiag_Ctrl_24/2
  MOD_OutputDiag_Ctrl_24/1 -> Switch4/2
  GT5/1(y) -> MOD_OutputDiag_Ctrl_24/1
  [boOut25Diag] -> MOD_OutputDiag_Ctrl_25/2
  [boCtrlValid] -> MOD_OutputDiag_Ctrl_25/3
  MOD_OutputDiag_Ctrl_25/1 -> Switch5/2
  Constant13/1 -> GT6/2(u2)
  GT6/1(y) -> MOD_OutputDiag_Ctrl_25/1
  [boCtrlValid] -> MOD_OutputDiag_Ctrl_26/3
  GT7/1(y) -> MOD_OutputDiag_Ctrl_26/1
  [boOut26Diag] -> MOD_OutputDiag_Ctrl_26/2
  Constant14/1 -> GT7/2(u2)
  MOD_OutputDiag_Ctrl_26/1 -> Switch6/2
  [boOut27Diag] -> MOD_OutputDiag_Ctrl_27/2
  GT8/1(y) -> MOD_OutputDiag_Ctrl_27/1
  [boCtrlValid] -> MOD_OutputDiag_Ctrl_27/3
  Constant15/1 -> GT8/2(u2)
  MOD_OutputDiag_Ctrl_27/1 -> Switch7/2
